simulink model "ScriptDemo"  (R2022b)
settings: configuration reference "TmVcThermal_Configuration_sub" (kept outside this file)
undefined symbols (not defined in the file or in its folder): aaaa, bbbb, cTmComprCtrl_D_u8HvacFlowTable_db, cTmComprCtrl_D_u8HvacFlowTable_sw, cTmComprCtrl_n_i16ChillCmpIMax, cTmComprCtrl_n_i16ChillCmpIMin, cTmComprCtrl_n_i16ChillCmpIMin666, cTmComprCtrl_n_i16ChillCmpPMax, cTmComprCtrl_n_i16ChillCmpPMin, cTmComprCtrl_n_i16CmpChillCoolRpmKiMax, cTmComprCtrl_n_i16CmpChillCoolRpmKiMin, cTmComprCtrl_n_i16CmpChillCoolRpmKpMax, cTmComprCtrl_n_i16CmpChillCoolRpmKpMin, cTmComprCtrl_n_i16CmpCoolRpmKiMax, cTmComprCtrl_n_i16CmpCoolRpmKiMin, cTmComprCtrl_n_i16CmpCoolRpmKpMax, cTmComprCtrl_n_i16CmpCoolRpmKpMin, cTmComprCtrl_n_i16SM4CmpHeatKiMax, cTmComprCtrl_n_i16SM4CmpHeatKiMin, cTmComprCtrl_n_i16SM4CmpHeatKpMax, cTmComprCtrl_n_i16SM4CmpHeatKpMin, cTmComprCtrl_n_i16SM5CmpHeatKiMax, cTmComprCtrl_n_i16SM5CmpHeatKiMin, cTmComprCtrl_n_i16SM5CmpHeatKpMax, cTmComprCtrl_n_i16SM5CmpHeatKpMin, cTmComprCtrl_n_i16SM6CmpHeatKiMax, cTmComprCtrl_n_i16SM6CmpHeatKiMin, cTmComprCtrl_n_i16SM6CmpHeatKpMax, cTmComprCtrl_n_i16SM6CmpHeatKpMin, cTmComprCtrl_n_u16CmpMaxSpdFanFltLimt, cTmComprCtrl_n_u16CmpMaxSpdLoSidePFltLimt, cTmComprCtrl_n_u16CmpMaxSpdSensorFltLimt, cTmComprCtrl_n_u16CompMinRpm, cTmComprCtrl_n_u16CompRpmIncThres, cTmComprCtrl_t_u16BattCooltFFPeriod, cTmComprCtrl_t_u16BattCooltPIPeriod, cTmComprCtrl_t_u16CmpCoolFFPeriod, cTmComprCtrl_t_u16CmpCoolPIPeriod, cTmComprCtrl_t_u16CoolCmpChillFFPeriod, cTmComprCtrl_t_u16CoolCmpChillPIPeriod, cTmComprCtrl_t_u16SM4CmpHeatFFPeriod, cTmComprCtrl_t_u16SM4CmpHeatPIPeriod, cTmComprCtrl_t_u16SM5CmpHeatFFPeriod, cTmComprCtrl_t_u16SM5CmpHeatPIPeriod, cTmComprCtrl_t_u16SM6CmpHeatFFPeriod, cTmComprCtrl_t_u16SM6CmpHeatPIPeriod, cTmComprCtrl_Te_EvapClearInteg, cTmComprCtrl_Te_i16HpReqTempSaturoffset, cTmComprCtrl_Te_i16SatLpReplaceDiff, cTmComprCtrl_Te_i16SM3BatDiffStartEvapDecOffset, cTmComprCtrl_Te_i16SM3EvapLo, cTmComprCtrl_Te_i16SM3TBatDiffEntEvapDecOffset, cTmComprCtrl_Te_i16SM3TBatDiffEntEvapDecOffsetQuit, cTmComprCtrl_Te_s32ErrCmpChillPIContinueCoolH, cTmComprCtrl_Te_s32ErrCmpChillPIContinueCoolL, cTmComprCtrl_Te_s32ErrCmpPIContinueChillH, cTmComprCtrl_Te_s32ErrCmpPIContinueChillL, cTmComprCtrl_Te_s32ErrCmpPIContinueCoolH, cTmComprCtrl_Te_s32ErrCmpPIContinueCoolL, cTmComprCtrl_Te_s32ErrCmpPIContinueHeatH ... (+398)
libraries: simulink x846, PCMULib x711, simulink_need_slupdate x4
(part 7 of 49)

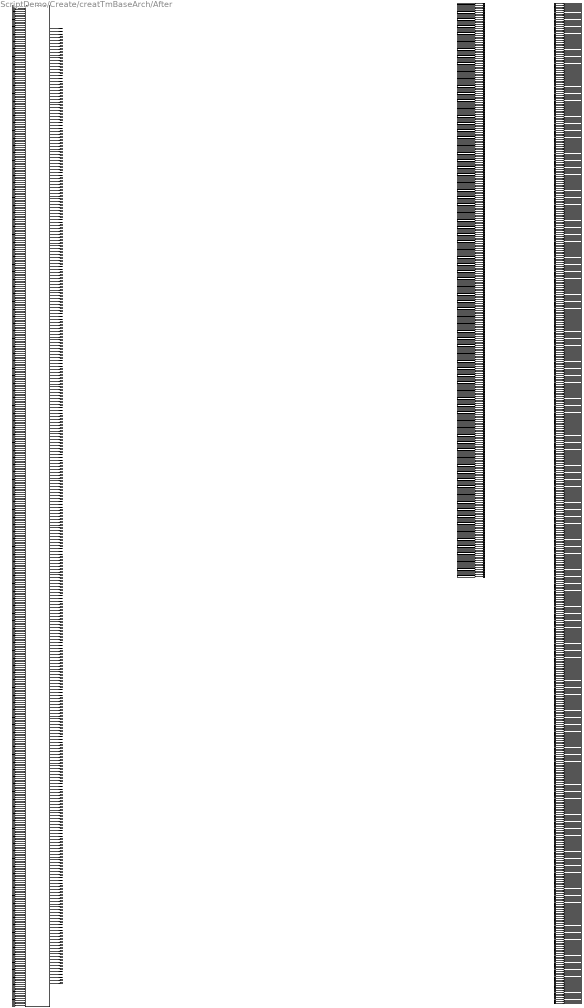
== system ScriptDemo/Create/creatTmBaseArch/After ==
  Ground{,1..567} (568 alike) : Ground
  Terminator{,1..325} (326 alike) : Terminator
  TmSwArch : ModelReference  ModelNameDialog=TmSwArch  ModelReferenceVersion=1.508
  wires:
  [sTmIn_L_s32WhlMotCooltFlowMinReq] -> TmSwArch/1
  [sTmIn_Te_s32WhlMotSysCooltT] -> TmSwArch/2
  [sTmIn_D_u8EradCoolReq] -> TmSwArch/3
  [sTmIn_Te_s32EradInvActl] -> TmSwArch/4
  [sTmIn_Te_s32EradWndgActl] -> TmSwArch/5
  [sTmIn_Tq_s32WhlMotSysTqEst] -> TmSwArch/6
  [sTmIn_D_u8DcdcCoolReq] -> TmSwArch/7
  [sTmIn_Te_s32DcdcActl] -> TmSwArch/8
  [sTmIn_L_s32DcDcMinCooltFlow] -> TmSwArch/9
  [sTmIn_D_u8ObcCoolReq] -> TmSwArch/10
  [sTmIn_D_u8OnBdChrgrHndlSts] -> TmSwArch/11
  [sTmIn_Te_s32ObcActl] -> TmSwArch/12
  [sTmIn_L_s32OnBdChrgrMinCooltFlow] -> TmSwArch/13
  [sTmIn_Te_s32OnBdChrgrCooltT] -> TmSwArch/14
  [sTmIn_Te_s32TDcDcCoolt] -> TmSwArch/15
  [sTmIn_D_u8HvBattCooltLvl] -> TmSwArch/16
  [sTmIn_D_u8DCChrgnHndlSts] -> TmSwArch/17
  [sTmIn_D_u8HvBattCoolgReq] -> TmSwArch/18
  [sTmIn_D_u8HvBattHeatgReq] -> TmSwArch/19
  [sTmIn_D_u8HvBattThermReq] -> TmSwArch/20
  [sTmIn_D_u16HVvBattLimnIndcn] -> TmSwArch/21
  [sTmIn_Pw_s32HvBattClimaPwr] -> TmSwArch/22
  [sTmIn_Te_s32BattHv] -> TmSwArch/23
  [sTmIn_Te_s32HvBattCooltT] -> TmSwArch/24
  [sTmIn_Te_s32HvBattCooltTReq] -> TmSwArch/25
  [sTmIn_L_s32HvBattCoolFlow1] -> TmSwArch/26
  [sTmIn_Te_s32HvBattCooltTOut] -> TmSwArch/27
  [sTmIn_L_s32IsgCooltFlowMinReq] -> TmSwArch/28
  [sTmIn_Te_s32Coolt] -> TmSwArch/29
  [sTmIn_D_u8HvgCoolReq] -> TmSwArch/30
  [sTmIn_Te_s32HvgInvActl] -> TmSwArch/31
  [sTmIn_Te_s32HvgWndgActl] -> TmSwArch/32
  [sTmIn_D_u8EngCooltLvl] -> TmSwArch/33
  [sTmIn_U_s32Sys] -> TmSwArch/34
  [sTmIn_D_u8UsgModSts1WdSts] -> TmSwArch/35
  [sTmIn_D_u8LVPwrSplyErrSts] -> TmSwArch/36
  [sTmIn_Z_s32RoadIncln] -> TmSwArch/37
  [sTmIn_D_u8CarModSts1] -> TmSwArch/38
  [sTmIn_Te_s32AmbTEstimd] -> TmSwArch/39
  [sTmIn_Te_s32Evap] -> TmSwArch/40
  [sTmIn_Te_s32EvapReq] -> TmSwArch/41
  [sTmIn_Te_s32HeadEstimdFirstRow] -> TmSwArch/42
  [sTmIn_Te_s32HeatrAirTReq] -> TmSwArch/43
  [sTmIn_Te_s32HvacHexAirT] -> TmSwArch/44
  [sTmIn_X_s32ClimtRcirc] -> TmSwArch/45
  [sTmIn_md_s32HexHeatrAirMFlowEstimd] -> TmSwArch/46
  [sTmIn_md_s32HvacAirMFlowEstimd] -> TmSwArch/47
  [yTmIn_B_AirCondEnbl] -> TmSwArch/48
  [yTmIn_B_ClimaDefrstSts] -> TmSwArch/49
  [yTmIn_B_HvacHeatgReq] -> TmSwArch/50
  [sTmIn_Te_s32IncarTemp] -> TmSwArch/51
  [yTmIn_B_AmbTEstimdQf] -> TmSwArch/52
  [sTmIn_D_u8IncarTempQf] -> TmSwArch/53
  [yTmIn_B_HvacOsaAndRecActrQfForHp] -> TmSwArch/54
  [yTmIn_B_TeEvap] -> TmSwArch/55
  [yTmIn_B_HvacHexAirTQf] -> TmSwArch/56
  [sTmIn_D_u8HvacFanSts] -> TmSwArch/57
  [yTmIn_B_ImpactDetect] -> TmSwArch/58
  [yTmIn_B_BattPmpOPflg] -> TmSwArch/59
  [yTmIn_B_BattPmpOPTF] -> TmSwArch/60
  [yTmIn_B_BattPmpSBflg] -> TmSwArch/61
  [yTmIn_B_BattPmpSBTF] -> TmSwArch/62
  [yTmIn_B_BattPmpSGflg] -> TmSwArch/63
  [yTmIn_B_BattPmpSGTF] -> TmSwArch/64
  [yTmIn_B_EmotPmpOPflg] -> TmSwArch/65
  [yTmIn_B_EmotPmpOPTF] -> TmSwArch/66
  [yTmIn_B_EmotPmpSBflg] -> TmSwArch/67
  [yTmIn_B_EmotPmpSBTF] -> TmSwArch/68
  [yTmIn_B_EmotPmpSGflg] -> TmSwArch/69
  [yTmIn_B_EmotPmpSGTF] -> TmSwArch/70
  [yTmIn_B_FanOutOPflg] -> TmSwArch/71
  [yTmIn_B_FanOutOPTF] -> TmSwArch/72
  [yTmIn_B_FanOutSBflg] -> TmSwArch/73
  [yTmIn_B_FanOutSBTF] -> TmSwArch/74
  [yTmIn_B_FanOutSGflg] -> TmSwArch/75
  [yTmIn_B_FanOutSGTF] -> TmSwArch/76
  [yTmIn_B_HmPumpOCflg] -> TmSwArch/77
  [yTmIn_B_HmPumpOCTF] -> TmSwArch/78
  [yTmIn_B_HmPumpSBflg] -> TmSwArch/79
  [yTmIn_B_HmPumpSBTF] -> TmSwArch/80
  [yTmIn_B_HmPumpSGflg] -> TmSwArch/81
  [yTmIn_B_HmPumpSGTF] -> TmSwArch/82
  [yTmIn_B_Sov1OPTF] -> TmSwArch/83
  [yTmIn_B_Sov1OPflg] -> TmSwArch/84
  [yTmIn_B_Sov1SBTF] -> TmSwArch/85
  [yTmIn_B_Sov1SBflg] -> TmSwArch/86
  [yTmIn_B_Sov1SGTF] -> TmSwArch/87
  [yTmIn_B_Sov1SGflg] -> TmSwArch/88
  [yTmIn_B_Sov2OPTF] -> TmSwArch/89
  [yTmIn_B_Sov2OPflg] -> TmSwArch/90
  [yTmIn_B_Sov2SBTF] -> TmSwArch/91
  [yTmIn_B_Sov2SBflg] -> TmSwArch/92
  [yTmIn_B_Sov2SGTF] -> TmSwArch/93
  [yTmIn_B_Sov2SGflg] -> TmSwArch/94
  [yTmIn_B_Sov3OPTF] -> TmSwArch/95
  [yTmIn_B_Sov3OPflg] -> TmSwArch/96
  [yTmIn_B_Sov3SBTF] -> TmSwArch/97
  [yTmIn_B_Sov3SBflg] -> TmSwArch/98
  [yTmIn_B_Sov3SGTF] -> TmSwArch/99
  [yTmIn_B_Sov3SGflg] -> TmSwArch/100
  [yTmIn_B_Sov4OPTF] -> TmSwArch/101
  [yTmIn_B_Sov4OPflg] -> TmSwArch/102
  [yTmIn_B_Sov4SBTF] -> TmSwArch/103
  [yTmIn_B_Sov4SBflg] -> TmSwArch/104
  [yTmIn_B_Sov4SGTF] -> TmSwArch/105
  [yTmIn_B_Sov4SGflg] -> TmSwArch/106
  [yTmIn_B_Sov5OPTF] -> TmSwArch/107
  [yTmIn_B_Sov5OPflg] -> TmSwArch/108
  [yTmIn_B_Sov5SBTF] -> TmSwArch/109
  [yTmIn_B_Sov5SBflg] -> TmSwArch/110
  [yTmIn_B_Sov5SGTF] -> TmSwArch/111
  [yTmIn_B_Sov5SGflg] -> TmSwArch/112
  [sTmIn_X_s32BattCooltPmpReq2F] -> TmSwArch/113
  [sTmIn_X_s32PTCPumpSpdReq2F] -> TmSwArch/114
  [sTmIn_D_u8CmprStsEnaReq2F] -> TmSwArch/115
  [sTmIn_n_s32CmprSpdReq2F] -> TmSwArch/116
  [sTmIn_Pw_s32CmprPwrEnaReq2F] -> TmSwArch/117
  [sTmIn_D_u8GrlShttrTrqBstReq2F] -> TmSwArch/118
  [sTmIn_D_u8BcfvVlvRefReq2F] -> TmSwArch/119
  [sTmIn_X_u8BcfvVlvPosReq2F] -> TmSwArch/120
  [sTmIn_D_u8BctvVlvRefReq2F] -> TmSwArch/121
  [sTmIn_X_u8BctvVlvPosReq2F] -> TmSwArch/122
  [yTmIn_B_BExvCalReq2F] -> TmSwArch/123
  [yTmIn_B_BExvMoveEnReq2F] -> TmSwArch/124
  [sTmIn_X_s32BExvPosnReq2F] -> TmSwArch/125
  [yTmIn_B_CExvCalReq2F] -> TmSwArch/126
  [yTmIn_B_CExvMoveEnaReq2F] -> TmSwArch/127
  [sTmIn_X_s32CExvPosnReq2F] -> TmSwArch/128
  [yTmIn_B_EctvVlvMoveEnaReq2F] -> TmSwArch/129
  [sTmIn_X_u8EctvVlvPosReq2F] -> TmSwArch/130
  [yTmIn_B_EExvCalReq2F] -> TmSwArch/131
  [yTmIn_B_EExvMoveEnaReq2F] -> TmSwArch/132
  [sTmIn_X_s32EExvPosnReq2F] -> TmSwArch/133
  [yTmIn_B_PtcEnaReq2F] -> TmSwArch/134
  [sTmIn_Pw_s32PtcPwrReq2F] -> TmSwArch/135
  [sTmIn_Te_s32PtcTReq2F] -> TmSwArch/136
  [sTmIn_L_s32PtcFlowReq2F] -> TmSwArch/137
  [sTmIn_X_s32FanPwmReq2F] -> TmSwArch/138
  [sTmIn_Z_s32VaneCtrlAngleReq2F] -> TmSwArch/139
  [sTmIn_X_s32EmCooltPmpReq2F] -> TmSwArch/140
  [yTmIn_B_HpmSov1ActvCmd2F] -> TmSwArch/141
  [yTmIn_B_HpmSov2ActvCmd2F] -> TmSwArch/142
  [yTmIn_B_HpmSov3ActvCmd2F] -> TmSwArch/143
  [yTmIn_B_EvaprVlvReqFrnt2F] -> TmSwArch/144
  [yTmIn_B_ChillerValveReq2F] -> TmSwArch/145
  [yTmIn_B_VaneCalEnbl2F] -> TmSwArch/146
  [yTmIn_B_HpmSov1Actv2FReq] -> TmSwArch/147
  [yTmIn_B_HpmSov2Actv2FReq] -> TmSwArch/148
  [yTmIn_B_HpmSov3Actv2FReq] -> TmSwArch/149
  [yTmIn_B_BattPmp2FReq] -> TmSwArch/150
  [yTmIn_B_PTCPumpSpd2FReq] -> TmSwArch/151
  [yTmIn_B_EvaprVlvFrnt2FReq] -> TmSwArch/152
  [yTmIn_B_CmprPwrEna2FReq] -> TmSwArch/153
  [yTmIn_B_CmprSpd2FReq] -> TmSwArch/154
  [yTmIn_B_CmprStsEna2FReq] -> TmSwArch/155
  [yTmIn_B_GrlShttrTrqBst2FReq] -> TmSwArch/156
  [yTmIn_B_BcfvVlvPos2FReq] -> TmSwArch/157
  [yTmIn_B_BcfvVlvRef2FReq] -> TmSwArch/158
  [yTmIn_B_BctvVlvPos2FReq] -> TmSwArch/159
  [yTmIn_B_BctvVlvRef2FReq] -> TmSwArch/160
  [yTmIn_B_BExvCal2FReq] -> TmSwArch/161
  [yTmIn_B_BExvMoveEna2FReq] -> TmSwArch/162
  [yTmIn_B_BExvPosn2FReq] -> TmSwArch/163
  [yTmIn_B_CExvCal2FReq] -> TmSwArch/164
  [yTmIn_B_CExvMoveEna2FReq] -> TmSwArch/165
  [yTmIn_B_CExvPosn2FReq] -> TmSwArch/166
  [yTmIn_B_ChillerValve2FReq] -> TmSwArch/167
  [yTmIn_B_EctvVlvMoveEna2FReq] -> TmSwArch/168
  [yTmIn_B_EctvVlvPos2FReq] -> TmSwArch/169
  [yTmIn_B_EExvCal2FReq] -> TmSwArch/170
  [yTmIn_B_EExvMoveEna2FReq] -> TmSwArch/171
  [yTmIn_B_EExvPosn2FReq] -> TmSwArch/172
  [yTmIn_B_PtcEna2FReq] -> TmSwArch/173
  [yTmIn_B_PtcFlow2FReq] -> TmSwArch/174
  [yTmIn_B_PtcPwr2FReq] -> TmSwArch/175
  [yTmIn_B_PtcT2FReq] -> TmSwArch/176
  [yTmIn_B_FanPwm2FReq] -> TmSwArch/177
  [yTmIn_B_VaneCalEnbl2FReq] -> TmSwArch/178
  [yTmIn_B_VaneCtrlAngle2FReq] -> TmSwArch/179
  [yTmIn_B_EmCooltPmp2FReq] -> TmSwArch/180
  [sTmIn_D_u8AcCmpr] -> TmSwArch/181
  [sTmIn_D_u8BattCoolLelIn] -> TmSwArch/182
  [sTmIn_D_u8EldtCoolLelIn] -> TmSwArch/183
  [sTmIn_D_u8ForHvacTyp] -> TmSwArch/184
  [sTmIn_D_u8HeatPump] -> TmSwArch/185
  [sTmIn_D_u8HvacRe] -> TmSwArch/186
  [sTmIn_D_u8Refrigerant] -> TmSwArch/187
  [sTmIn_D_u8ShutterConfig] -> TmSwArch/188
  [sTmIn_U_s32AcCompDischrgT] -> TmSwArch/189
  [sTmIn_U_s32AcCompInletT] -> TmSwArch/190
  [sTmIn_U_s32AcCondOutT] -> TmSwArch/191
  [sTmIn_U_s32AcEvapOutT] -> TmSwArch/192
  [sTmIn_U_s32AcIntelCondOutT] -> TmSwArch/193
  [sTmIn_U_s32HiSideP] -> TmSwArch/194
  [sTmIn_U_s32HiSidePNHP] -> TmSwArch/195
  [sTmIn_U_s32LoSideP] -> TmSwArch/196
  [sTmIn_U_s32CooltTSigForDtElec] -> TmSwArch/197
  [yTmIn_B_CPSRFbSt] -> TmSwArch/198
  [sTmIn_U_s32BattVolt] -> TmSwArch/199
  [yTmIn_B_HvBattThermModUD] -> TmSwArch/200
  [sTmIn_D_u8EexvBlkErr] -> TmSwArch/201
  [sTmIn_D_u8EexvElecStsErr] -> TmSwArch/202
  [sTmIn_D_u8EexvNVMFlt] -> TmSwArch/203
  [sTmIn_D_u8EexvOvrTempErr] -> TmSwArch/204
  [sTmIn_D_u8EexvVoltgRangErr] -> TmSwArch/205
  [sTmIn_D_u8EexvOvrTrvlErr] -> TmSwArch/206
  [sTmIn_D_u8CexvBlkErr] -> TmSwArch/207
  [sTmIn_D_u8CexvElecStsErr] -> TmSwArch/208
  [sTmIn_D_u8CexvNVMFlt] -> TmSwArch/209
  [sTmIn_D_u8CexvOvrTempErr] -> TmSwArch/210
  [sTmIn_D_u8CexvVoltgRangErr] -> TmSwArch/211
  [sTmIn_D_u8CexvOvrTrvlErr] -> TmSwArch/212
  [sTmIn_D_u8EctvFaultSts] -> TmSwArch/213
  [sTmIn_D_u8EctvTempSts] -> TmSwArch/214
  [sTmIn_D_u8EctvVoltSts] -> TmSwArch/215
  [sTmIn_D_u8BexvBlkErr] -> TmSwArch/216
  [sTmIn_D_u8BexvCalibSts] -> TmSwArch/217
  [sTmIn_D_u8BexvElecStsErr] -> TmSwArch/218
  [sTmIn_D_u8BexvNVMFlt] -> TmSwArch/219
  [sTmIn_D_u8BexvOvrTempErr] -> TmSwArch/220
  [sTmIn_D_u8BexvOvrTrvlErr] -> TmSwArch/221
  [sTmIn_D_u8BexvPreHeatgSts] -> TmSwArch/222
  [sTmIn_D_u8BexvVoltgRangErr] -> TmSwArch/223
  [sTmIn_X_s32BexvPosSts] -> TmSwArch/224
  [yTmIn_B_BexvComFault] -> TmSwArch/225
  [sTmIn_D_u8BcfvFaultSts] -> TmSwArch/226
  [sTmIn_D_u8BcfvNVMFlt] -> TmSwArch/227
  [sTmIn_D_u8BcfvTempSts] -> TmSwArch/228
  [sTmIn_D_u8BcfvVoltSts] -> TmSwArch/229
  [sTmIn_D_u8BctvFaultSts] -> TmSwArch/230
  [sTmIn_D_u8BctvNVMFlt] -> TmSwArch/231
  [sTmIn_D_u8BctvTempSts] -> TmSwArch/232
  [sTmIn_D_u8BctvVoltSts] -> TmSwArch/233
  [sTmIn_X_s32BctvPosSts] -> TmSwArch/234
  [sTmIn_D_u8CmprRAMFault] -> TmSwArch/235
  [sTmIn_D_u8CmprROMFault] -> TmSwArch/236
  [sTmIn_D_u8CmprRotorLockStat] -> TmSwArch/237
  [sTmIn_D_u8CmprSts1] -> TmSwArch/238
  [sTmIn_D_u8HVoltResonanceStat] -> TmSwArch/239
  [sTmIn_D_u8InCurrOverCurrStat] -> TmSwArch/240
  [sTmIn_D_u8LiquidSluggingStat] -> TmSwArch/241
  [sTmIn_D_u8MotorCurrOverCurrStat] -> TmSwArch/242
  [sTmIn_D_u8OverMotorCurrStat] -> TmSwArch/243
  [sTmIn_D_u8OverPowerStat] -> TmSwArch/244
  [sTmIn_I_s32ElacCmprHvActl] -> TmSwArch/245
  [sTmIn_n_s32ElacCmprActl] -> TmSwArch/246
  [sTmIn_Te_s32CmprT1] -> TmSwArch/247
  [sTmIn_U_s32ElacCmprHvActl] -> TmSwArch/248
  [sTmIn_D_u8ErrRespAGM] -> TmSwArch/249
  [sTmIn_D_u8GrlActTrqBoost] -> TmSwArch/250
  [sTmIn_D_u8GrlHldTrqActive] -> TmSwArch/251
  [sTmIn_D_u8GrlShttrMoveActive] -> TmSwArch/252
  [sTmIn_D_u8GrlShttrNVMFlt] -> TmSwArch/253
  [sTmIn_D_u8GrlShttrOvertravelErr] -> TmSwArch/254
  [sTmIn_D_u8GrlShttrOverVolt] -> TmSwArch/255
  [sTmIn_D_u8GrlShttrStsShttrActrFlt] -> TmSwArch/256
  [sTmIn_D_u8GrlShttrStsShttrBlkd] -> TmSwArch/257
  [sTmIn_D_u8GrlShttrStsShttrCalActv] -> TmSwArch/258
  [sTmIn_D_u8GrlShttrStsShttrCalIndcd] -> TmSwArch/259
  [sTmIn_D_u8GrlShttrStsShttrElecErr] -> TmSwArch/260
  [sTmIn_D_u8GrlShttrStsShttrSnsrFlt] -> TmSwArch/261
  [sTmIn_D_u8GrlShttrStsShttrTErr] -> TmSwArch/262
  [sTmIn_D_u8GrlShttrStsShttrULoErr] -> TmSwArch/263
  [sTmIn_X_s32GrlShttrStsShttrPosnRaw] -> TmSwArch/264
  [sTmIn_D_u8CircForDrvrShoOrOpen] -> TmSwArch/265
  [sTmIn_D_u8CooltTInSnsrFlt] -> TmSwArch/266
  [sTmIn_D_u8CooltTOutOfRng] -> TmSwArch/267
  [sTmIn_D_u8CooltTOutSnsrFlt] -> TmSwArch/268
  [sTmIn_D_u8HeatrStsSig] -> TmSwArch/269
  [sTmIn_D_u8HvOutOfRng] -> TmSwArch/270
  [sTmIn_D_u8ICnsOutOfRng] -> TmSwArch/271
  [sTmIn_D_u8MemErr] -> TmSwArch/272
  [sTmIn_D_u8SelfTmpSigHwProtn] -> TmSwArch/273
  [sTmIn_D_u8SelfTmpSigOvrheatg] -> TmSwArch/274
  [sTmIn_D_u8TInMtrlSnsrFlt] -> TmSwArch/275
  [sTmIn_D_u8ULoOutOfRng] -> TmSwArch/276
  [sTmIn_Pw_s32HvHeatrPwrCns] -> TmSwArch/277
  [sTmIn_Pw_s32HvHeatrPwrCnsDes] -> TmSwArch/278
  [sTmIn_Te_s32WtrTInIntk] -> TmSwArch/279
  [sTmIn_Te_s32WtrTInOutl] -> TmSwArch/280
  [sTmIn_D_u8SrvRqrd] -> TmSwArch/281
  [sTmIn_D_u8TmpSigProtnOfSelfTmp] -> TmSwArch/282
  [sTmIn_D_u8HvCoolgCmd] -> TmSwArch/283
  [sTmIn_D_u8HvHvacCmd] -> TmSwArch/284
  [sTmIn_D_u8HvActvSts] -> TmSwArch/285
  [sTmIn_D_u8PowerPackStatus] -> TmSwArch/286
  [sTmIn_Pw_s32HvCoolgAllwd] -> TmSwArch/287
  [sTmIn_Pw_s32HvHeatgAllwd] -> TmSwArch/288
  [yTmIn_B_ElAcEnable] -> TmSwArch/289
  [yTmIn_B_HvCooltHeatrEnad] -> TmSwArch/290
  [sTmIn_v_s32VehSpdLgt] -> TmSwArch/291
  [yTmIn_B_StarDiagEval] -> TmSwArch/292
  [sTmIn_D_u8HvActvReq] -> TmSwArch/293
  [sTmIn_D_u8DCChrgSt] -> TmSwArch/294
  [yTmIn_B_NOPCoolReq] -> TmSwArch/295
  [sTmIn_Pw_s32HvBattChrgnPwrCritDes1] -> TmSwArch/296
  [yTmIn_B_ChargePsr] -> TmSwArch/297
  [sTmIn_Te_s32BattHvMin] -> TmSwArch/298
  [sTmIn_D_u8HvBattSupChrgThermSts] -> TmSwArch/299
  [sTmIn_D_u8OnBdChrgrSt] -> TmSwArch/300
  [sTmIn_D_u8DistHvBatt] -> TmSwArch/301
  [sTmIn_D_u8ElecDriveline] -> TmSwArch/302
  [sTmIn_D_u8HiWayAsst] -> TmSwArch/303
  [sTmIn_D_u8CruiseCtrl] -> TmSwArch/304
  [sTmIn_D_u8BattCntct] -> TmSwArch/305
  [sTmIn_U_s32HvBattUDc] -> TmSwArch/306
  [yTmIn_B_EvaprTFrntUD] -> TmSwArch/307
  [sTmIn_Te_s32HmiCmptmtTSpForRowFirstRi] -> TmSwArch/308
  [sTmIn_Te_s32HmiCmptmtTSpForRowFirstLe] -> TmSwArch/309
  [sTmIn_D_u8HvUSplyErrSts] -> TmSwArch/310
  [sTmIn_D_u8LnchModSts] -> TmSwArch/311
  [sTmIn_D_u8LaunchCtrl] -> TmSwArch/312
  [sTmIn_X_s32HvacTFlpActlPosnFrtRowLe] -> TmSwArch/313
  [sTmIn_X_s32HvacTFlpActlPosnFrtRowRi] -> TmSwArch/314
  [sTmIn_D_u8HmiCmptmtTSpSpclForRowFirstLe] -> TmSwArch/315
  [sTmIn_D_u8HmiCmptmtTSpSpclForRowFirstRi] -> TmSwArch/316
  [sTmIn_D_u8SysQf] -> TmSwArch/317
  [yTmIn_B_ErrRespHVCH] -> TmSwArch/318
  [sTmIn_I_s32HeatrICnsSig] -> TmSwArch/319
  [sTmIn_D_u8HeatrInfoCompProtn] -> TmSwArch/320
  [sTmIn_U_u8SplyUForCtrlUnitVal] -> TmSwArch/321
  [sTmIn_D_u8SelfSigProOfTmpResd] -> TmSwArch/322
  [sTmIn_D_u8ResdForSnsrFlt] -> TmSwArch/323
  [sTmIn_D_u8SrvRqrdResd] -> TmSwArch/324
  [sTmIn_D_u8FltInComHVCH] -> TmSwArch/325
  [sTmIn_D_u8FltPrsnt] -> TmSwArch/326
  [sTmIn_D_u8FltPrsntResd] -> TmSwArch/327
  [yTmIn_B_EctvComFault] -> TmSwArch/328
  [sTmIn_D_u8EctvPosSts] -> TmSwArch/329
  [sTmIn_D_u8EctvRunSts] -> TmSwArch/330
  [sTmIn_D_u8EctvSpdLvl] -> TmSwArch/331
  [yTmIn_B_BctvComFault] -> TmSwArch/332
  [sTmIn_D_u8BctvVlvMode] -> TmSwArch/333
  [sTmIn_D_u8BctvRunSts] -> TmSwArch/334
  [sTmIn_D_u8BctvSpdLvl] -> TmSwArch/335
  [yTmIn_B_BcfvComFault] -> TmSwArch/336
  [sTmIn_D_u8BcfvVlvMode] -> TmSwArch/337
  [sTmIn_X_s32BcfvPosSts] -> TmSwArch/338
  [sTmIn_D_u8BcfvRunSts] -> TmSwArch/339
  [sTmIn_D_u8BcfvSpdLvl] -> TmSwArch/340
  [sTmIn_D_u8ErrRespACCM] -> TmSwArch/341
  [sTmIn_D_u8SpdErrSts] -> TmSwArch/342
  [sTmIn_D_u8CtrlrErrSts] -> TmSwArch/343
  [sTmIn_D_u8AccmDrvrSircSnErrStsts] -> TmSwArch/344
  [sTmIn_D_u8DrvrSircSnstPlausErrSts] -> TmSwArch/345
  [sTmIn_D_u8AccmHvSnsrU1ErrSts] -> TmSwArch/346
  [sTmIn_D_u8AccmHvSnsrU2ErrSts] -> TmSwArch/347
  [sTmIn_D_u8AccmHvSnsrIErrSts] -> TmSwArch/348
  [sTmIn_D_u8AccmSnsrICrctErrSts] -> TmSwArch/349
  [sTmIn_D_u8HvSnsrIPlausErrSts] -> TmSwArch/350
  [sTmIn_D_u8HvSnsrUPlausErrSts] -> TmSwArch/351
  [sTmIn_D_u8AccmPhaseWireErrSts] -> TmSwArch/352
  [sTmIn_D_u8AccmT1ErrSts] -> TmSwArch/353
  [sTmIn_D_u8AccmT2ErrSts] -> TmSwArch/354
  [sTmIn_D_u8AccmCmprTOperErr1] -> TmSwArch/355
  [sTmIn_D_u8AccmCmprTOperErr2] -> TmSwArch/356
  [sTmIn_D_u8TPlausErrSts] -> TmSwArch/357
  [sTmIn_D_u8AccmLoUSplyErrSts] -> TmSwArch/358
  [sTmIn_I_s32CmprFbCmprIPha] -> TmSwArch/359
  [sTmIn_D_u8CmprSts2] -> TmSwArch/360
  [sTmIn_Te_s32CmprT2] -> TmSwArch/361
  [sTmIn_D_u8EEPROMFault] -> TmSwArch/362
  [sTmIn_D_u8LostCommStat] -> TmSwArch/363
  [sTmIn_D_u8CmprSpdIncrReq] -> TmSwArch/364
  [sTmIn_D_u8BexvMovSts] -> TmSwArch/365
  [yTmIn_B_CexvComFault] -> TmSwArch/366
  [sTmIn_X_s32CexvPosSts] -> TmSwArch/367
  [sTmIn_D_u8CexvCalibSts] -> TmSwArch/368
  [sTmIn_D_u8CexvMovSts] -> TmSwArch/369
  [sTmIn_D_u8CexvPreHeatgSts] -> TmSwArch/370
  [yTmIn_B_EexvComFault] -> TmSwArch/371
  [sTmIn_X_s32EexvPosSts] -> TmSwArch/372
  [sTmIn_D_u8EexvCalibSts] -> TmSwArch/373
  [sTmIn_D_u8EexvMovSts] -> TmSwArch/374
  [sTmIn_D_u8EexvPreHeatgSts] -> TmSwArch/375
  [yTmIn_B_HvacHexAirTUD] -> TmSwArch/376
  [yTmIn_B_EcoClimaSts] -> TmSwArch/377
  [sTmIn_t_s32BattPmpPwmTHigh] -> TmSwArch/378
  [yTmIn_B_BattPmpTHighValid] -> TmSwArch/379
  [sTmIn_t_s32BattPmpPwmTLow] -> TmSwArch/380
  [yTmIn_B_BattPmpTLowValid] -> TmSwArch/381
  [sTmIn_t_s32EmotPmpPwmTHigh] -> TmSwArch/382
  [yTmIn_B_EmotPmpTHighValid] -> TmSwArch/383
  [sTmIn_t_s32EmotPmpPwmTLow] -> TmSwArch/384
  [yTmIn_B_EmotPmpTLowValid] -> TmSwArch/385
  [sTmIn_t_s32FanPwmTHigh] -> TmSwArch/386
  [yTmIn_B_FanTHighValid] -> TmSwArch/387
  [sTmIn_t_s32FanPwmTLow] -> TmSwArch/388
  [yTmIn_B_FanTLowValid] -> TmSwArch/389
  [sTmIn_t_s32HmPumpPwmTHigh] -> TmSwArch/390
  [yTmIn_B_HmPumpTHighValid] -> TmSwArch/391
  [sTmIn_t_s32HmPumpPwmTLow] -> TmSwArch/392
  [yTmIn_B_HmPumpTLowValid] -> TmSwArch/393
  [sTmIn_D_u8HeatStopReq] -> TmSwArch/394
  [yTmIn_B_AD4CoolReq] -> TmSwArch/395
  [sTmIn_L_s32AD4CooltFlowReq] -> TmSwArch/396
  [sTmIn_L_s32DHUCooltFlowMinReq] -> TmSwArch/397
  [sTmIn_D_u8VcEvLoSidePOP] -> TmSwArch/398
  [sTmIn_D_u8VcEvLoSidePSB] -> TmSwArch/399
  [sTmIn_D_u8VcEvHiSidePOP] -> TmSwArch/400
  [sTmIn_D_u8VcEvHiSidePSB] -> TmSwArch/401
  [sTmIn_D_u8VcEvHiSideTmpSnrSG] -> TmSwArch/402
  [sTmIn_D_u8VcEvOutrCondOutTOP] -> TmSwArch/403
  [sTmIn_D_u8VcEvChillerOutTSG] -> TmSwArch/404
  [sTmIn_D_u8VcEvChillerOutTOP] -> TmSwArch/405
  [sTmIn_D_u8VcEvInrCondOutTSG] -> TmSwArch/406
  [sTmIn_D_u8VcEvInrCondOutTOP] -> TmSwArch/407
  [sTmIn_D_u8VcEvEvapOutTSG] -> TmSwArch/408
  [sTmIn_D_u8VcEvEvapOutTOP] -> TmSwArch/409
  [sTmIn_D_u8VcEvCmprDischrgTSG] -> TmSwArch/410
  [sTmIn_D_u8VcEvCmprDischrgTOP] -> TmSwArch/411
  [sTmIn_D_u8VcEvTmpClSrSG] -> TmSwArch/412
  [sTmIn_D_u8VcEvTmpClSrOP] -> TmSwArch/413
  [sTmIn_D_u8VcEvBattCooltLvlLo] -> TmSwArch/414
  [sTmIn_D_u8VcEvNoHpHighSidePSnrOP] -> TmSwArch/415
  [sTmIn_D_u8VcEvNoHpHighSidePSnrSB] -> TmSwArch/416
  [sTmIn_D_u8VcEvSov1OP] -> TmSwArch/417
  [sTmIn_D_u8VcEvSov1SB] -> TmSwArch/418
  [sTmIn_D_u8VcEvSov1SG] -> TmSwArch/419
  [sTmIn_D_u8VcEvSov2OP] -> TmSwArch/420
  [sTmIn_D_u8VcEvSov2SB] -> TmSwArch/421
  [sTmIn_D_u8VcEvSov2SG] -> TmSwArch/422
  [sTmIn_D_u8VcEvSov3OP] -> TmSwArch/423
  [sTmIn_D_u8VcEvSov3SB] -> TmSwArch/424
  [sTmIn_D_u8VcEvSov3SG] -> TmSwArch/425
  [sTmIn_D_u8VcEvSov4OP] -> TmSwArch/426
  [sTmIn_D_u8VcEvSov4SB] -> TmSwArch/427
  [sTmIn_D_u8VcEvSov4SG] -> TmSwArch/428
  [sTmIn_D_u8VcEvSov5OP] -> TmSwArch/429
  [sTmIn_D_u8VcEvSov5SB] -> TmSwArch/430
  [sTmIn_D_u8VcEvSov5SG] -> TmSwArch/431
  [sTmIn_D_u8VcEvSBFan] -> TmSwArch/432
  [sTmIn_D_u8VcEvSGFan] -> TmSwArch/433
  [sTmIn_D_u8VcEvOPFan] -> TmSwArch/434
  [sTmIn_D_u8VcEvFanOvrTShDwn] -> TmSwArch/435
  [sTmIn_D_u8VcEvBlokFan] -> TmSwArch/436
  [sTmIn_D_u8VcEvCircutInteFlt] -> TmSwArch/437
  [sTmIn_D_u8VcEvVolErrFan] -> TmSwArch/438
  [sTmIn_D_u8VcEvHmPumpSG] -> TmSwArch/439
  [sTmIn_D_u8VcEvHmPumpSB] -> TmSwArch/440
  [sTmIn_D_u8VcEvHmPumpOC] -> TmSwArch/441
  [sTmIn_D_u8VcEvHmPmpOvrTShutDwn] -> TmSwArch/442
  [sTmIn_D_u8VcEvHmPmpStall] -> TmSwArch/443
  [sTmIn_D_u8VcEvHmPmpVolErr] -> TmSwArch/444
  [sTmIn_D_u8VcEvHmPmpDyRn] -> TmSwArch/445
  [sTmIn_D_u8VcEvSGBatteryPmp] -> TmSwArch/446
  [sTmIn_D_u8VcEvSBBatteryPmp] -> TmSwArch/447
  [sTmIn_D_u8VcEvOCBatteryPmp] -> TmSwArch/448
  [sTmIn_D_u8VcEvBattPmpOvrTShutDwn] -> TmSwArch/449
  [sTmIn_D_u8VcEvBattPmpStall] -> TmSwArch/450
  [sTmIn_D_u8VcEvBattPmpVolErr] -> TmSwArch/451
  [sTmIn_D_u8VcEvBattPmpDyn] -> TmSwArch/452
  [sTmIn_D_u8VcEvSGEmotor] -> TmSwArch/453
  [sTmIn_D_u8VcEvSBEmotor] -> TmSwArch/454
  [sTmIn_D_u8VcEvOCEmotor] -> TmSwArch/455
  [sTmIn_D_u8VcEvEmPmpOvrTShutDwn] -> TmSwArch/456
  [sTmIn_D_u8VcEvEmPmpStall] -> TmSwArch/457
  [sTmIn_D_u8VcEvEmPmpVolErr] -> TmSwArch/458
  [sTmIn_D_u8VcEvEmPmpDyRn] -> TmSwArch/459
  [sTmIn_D_u8VcEvBctvOthrErr] -> TmSwArch/460
  [sTmIn_D_u8VcEvFltTemBCTV] -> TmSwArch/461
  [sTmIn_D_u8VcEvBctvBlk] -> TmSwArch/462
  [sTmIn_D_u8VcEvBctvErrResp] -> TmSwArch/463
  [sTmIn_D_u8VcEvFltVolBCTV] -> TmSwArch/464
  [sTmIn_D_u8VcEvBctvNVMFlt] -> TmSwArch/465
  [sTmIn_D_u8VcEvBctvIniFail] -> TmSwArch/466
  [sTmIn_D_u8VcEvBcfvOthrErr] -> TmSwArch/467
  [sTmIn_D_u8VcEvFltTempBCFV] -> TmSwArch/468
  [sTmIn_D_u8VcEvBcfvBlk] -> TmSwArch/469
  [sTmIn_D_u8VcEvBcfvErrResp] -> TmSwArch/470
  [sTmIn_D_u8VcEvFltVolBCFV] -> TmSwArch/471
  [sTmIn_D_u8VcEvBcfvNVMFlt] -> TmSwArch/472
  [sTmIn_D_u8VcEvBcfvIniFail] -> TmSwArch/473
  [sTmIn_D_u8VcEvEctvDrvMotorFlt] -> TmSwArch/474
  [sTmIn_D_u8VcEvWarnECRV] -> TmSwArch/475
  [sTmIn_D_u8VcEvEcrvErrResp] -> TmSwArch/476
  [sTmIn_D_u8VcEvFltVolECRV] -> TmSwArch/477
  [sTmIn_D_u8VcEvBexvIniFail] -> TmSwArch/478
  [sTmIn_D_u8VcEvBexvOvrTempErr] -> TmSwArch/479
  [sTmIn_D_u8VcEvBexvBlkErr] -> TmSwArch/480
  [sTmIn_D_u8VcEvBexvErrResp] -> TmSwArch/481
  [sTmIn_D_u8VcEvBexvVoltgRangErr] -> TmSwArch/482
  [sTmIn_D_u8VcEvBexvNVMFlt] -> TmSwArch/483
  [sTmIn_D_u8VcEvCexvIniFail] -> TmSwArch/484
  [sTmIn_D_u8VcEvCexvOvrTempErr] -> TmSwArch/485
  [sTmIn_D_u8VcEvCexvBlkErr] -> TmSwArch/486
  [sTmIn_D_u8VcEvCexvErrResp] -> TmSwArch/487
  [sTmIn_D_u8VcEvCexvVoltgRangErr] -> TmSwArch/488
  [sTmIn_D_u8VcEvCexvNVMFlt] -> TmSwArch/489
  [sTmIn_D_u8VcEvEexvIniFail] -> TmSwArch/490
  [sTmIn_D_u8VcEvEexvOvrTempErr] -> TmSwArch/491
  [sTmIn_D_u8VcEvEexvBlkErr] -> TmSwArch/492
  [sTmIn_D_u8VcEvEexvErrResp] -> TmSwArch/493
  [sTmIn_D_u8VcEvEexvVoltgRangErr] -> TmSwArch/494
  [sTmIn_D_u8VcEvEexvNVMFlt] -> TmSwArch/495
  [sTmIn_D_u8VcEvAccmUSplyErr] -> TmSwArch/496
  [sTmIn_D_u8VcEvAccmOCFlt] -> TmSwArch/497
  [sTmIn_D_u8VcEvAccmMotOvrCur] -> TmSwArch/498
  [sTmIn_D_u8VcEvAccmComFlt] -> TmSwArch/499
  [sTmIn_D_u8VcEvCurDrCirtACCM] -> TmSwArch/500
  [sTmIn_D_u8VcEvAccmRotorLock] -> TmSwArch/501
  [sTmIn_D_u8VcEvAccmOPFlt] -> TmSwArch/502
  [sTmIn_D_u8VcEvLiquidSluggingACCM] -> TmSwArch/503
  [sTmIn_D_u8VcEvMemFltAccm] -> TmSwArch/504
  [sTmIn_D_u8VcEvTM_AGM_OVRTEMP] -> TmSwArch/505
  [sTmIn_D_u8VcEvAgsBlk] -> TmSwArch/506
  [sTmIn_D_u8VcEvAgsErrResp] -> TmSwArch/507
  [sTmIn_D_u8VcEvAgsVoltErr] -> TmSwArch/508
  [sTmIn_D_u8VcEvAgsMechErr] -> TmSwArch/509
  [sTmIn_D_u8VcEvAgsNVMFlt] -> TmSwArch/510
  [sTmIn_D_u8VcEvAgsElecErr] -> TmSwArch/511
  [sTmIn_D_u8VcEvIGBTSpOrOpHVCH] -> TmSwArch/512
  [sTmIn_D_u8VcEvLoVoOvrHVCH] -> TmSwArch/513
  [sTmIn_D_u8VcEvVolMemErrHVCH] -> TmSwArch/514
  [sTmIn_D_u8VcEvComFltHVCH] -> TmSwArch/515
  [sTmIn_D_u8VcEvHiVoOvrHVCH] -> TmSwArch/516
  [sTmIn_D_u8VcEvCoolTempOutOfRng] -> TmSwArch/517
  [sTmIn_D_u8VcEvTempSerIntHVCH] -> TmSwArch/518
  [sTmIn_D_u8VcEvTempSerOutHVCH] -> TmSwArch/519
  [sTmIn_D_u8VcEvHWProtHVCH] -> TmSwArch/520
  [sTmIn_D_u8VcEvInterSerTempHVCH] -> TmSwArch/521
  [sTmIn_D_u8VcEvCurrOutOfRng] -> TmSwArch/522
  [sTmIn_D_u8LackRefrigerant] -> TmSwArch/523
  [sTmIn_D_u8HvBoostMod] -> TmSwArch/524
  [yTmIn_B_HmiMaxACReq] -> TmSwArch/525
  [yTmIn_B_GrlShttrAutoCalibReq2FReq] -> TmSwArch/526
  [yTmIn_B_GrlShttrAutoCalibReqReq2F] -> TmSwArch/527
  [sTmIn_X_s32PTCPumpPwmFb] -> TmSwArch/528
  [yTmIn_B_MessMissBctv] -> TmSwArch/529
  [yTmIn_B_MessMissBCFV] -> TmSwArch/530
  [yTmIn_B_MessMissECRV] -> TmSwArch/531
  [yTmIn_B_MessMissBEXV] -> TmSwArch/532
  [yTmIn_B_MessMissCEXV] -> TmSwArch/533
  [yTmIn_B_MessMissEEXV] -> TmSwArch/534
  [yTmIn_B_MessMissAccm] -> TmSwArch/535
  [yTmIn_B_MessMissAGM] -> TmSwArch/536
  [yTmIn_B_MessMissHVCH] -> TmSwArch/537
  [sTmIn_Tq_s32TotAxle] -> TmSwArch/538
  [sTmIn_Z_s32HvacModResp] -> TmSwArch/539
  [sTmIn_Te_s32HvBattTAvg] -> TmSwArch/540
  [yTmIn_B_AD4CoolReqForBkp] -> TmSwArch/541
  [sTmIn_L_s32AD4CooltFlowReqForBkp] -> TmSwArch/542
  [yTmIn_B_ChillerValveReqFb] -> TmSwArch/543
  [yTmIn_B_EvaprVlvReqFrntFb] -> TmSwArch/544
  [yTmIn_B_HpmSov1ActvCmdFb] -> TmSwArch/545
  [yTmIn_B_HpmSov2ActvCmdFb] -> TmSwArch/546
  [yTmIn_B_HpmSov3ActvCmdFb] -> TmSwArch/547
  [yTmIn_B_EmActivHeatAllwd] -> TmSwArch/548
  [sTmIn_D_u8IsgHeatFdBck] -> TmSwArch/549
  [sTmIn_D_u8WhlMotSysHeatFdBck] -> TmSwArch/550
  [sTmIn_Pw_s32IsgHeatPwrAct] -> TmSwArch/551
  [sTmIn_Pw_s32WhlMotSysHeatPwrAct] -> TmSwArch/552
  [sTmIn_Pw_s32ElecDrvHeatgPwrAllwd] -> TmSwArch/553
  [sTmIn_Pw_s32WhlMotSysHeatPwrMax] -> TmSwArch/554
  [sTmIn_Pw_s32IsgHeatPwrMax] -> TmSwArch/555
  [sTmIn_X_s32BattCooltPmpPwmFb] -> TmSwArch/556
  [sTmIn_D_u8CmprSupplrNo] -> TmSwArch/557
  [sTmIn_D_u8VcEvEctvBlk] -> TmSwArch/558
  [sTmIn_D_u8VcEvOVACCM] -> TmSwArch/559
  [sTmIn_D_u8VcEvAccmIgbtOvrTErr] -> TmSwArch/560
  [sTmIn_D_u8VcEvAccmSnsrFlt] -> TmSwArch/561
  [sTmIn_D_u8VcEvAccmPhaseFail] -> TmSwArch/562
  [yTmIn_B_AD4CoolReqForBkpUD] -> TmSwArch/563
  [yTmIn_B_AD4CoolReqUD] -> TmSwArch/564
  [yTmIn_B_AD4CooltFlowReqForBkpUD] -> TmSwArch/565
  [yTmIn_B_AD4CooltFlowReqUD] -> TmSwArch/566
  [sTmIn_D_u8VcEvOvrTempHVCH] -> TmSwArch/567
  [sTmIn_B_HvBattLimnIndcnUD] -> TmSwArch/568
  TmSwArch/1 -> [sTmOut_n_u16ElacCmprReq]
  TmSwArch/2 -> [sTmOut_D_u8ElacCmprRelease]
  TmSwArch/3 -> [sTmOut_Pw_s32ElacCmprMax]
  TmSwArch/4 -> [sTmOut_X_s32EexvVlvPosReq]
  TmSwArch/5 -> [yTmOut_B_EexvPosnCalibReq]
  TmSwArch/6 -> [yTmOut_B_EexvPosnMovEnable]
  TmSwArch/7 -> [sTmOut_X_s32BexvVlvPosReq]
  TmSwArch/8 -> [yTmOut_B_BexvPosnCalibReq]
  TmSwArch/9 -> [yTmOut_B_BexvPosnMovEnable]
  TmSwArch/10 -> [sTmOut_X_s32CexvVlvPosReq]
  TmSwArch/11 -> [yTmOut_B_CexvPosnCalibReq]
  TmSwArch/12 -> [yTmOut_B_CexvPosnMovEnable]
  TmSwArch/13 -> [sTmOut_D_u8BctvVlvRefDrvReq]
  TmSwArch/14 -> [sTmOut_X_u8BctvVlvPosReq]
  TmSwArch/15 -> [sTmOut_D_u8BcfvVlvRefDrvReq]
  TmSwArch/16 -> [sTmOut_X_u8BcfvVlvPosReq]
  TmSwArch/17 -> [yTmOut_B_EctvVlvMovEna]
  TmSwArch/18 -> [sTmOut_D_u8EctvVlvPosReq]
  TmSwArch/19 -> [sTmOut_Te_s32PTCTempReq]
  TmSwArch/20 -> [sTmOut_Z_s32PTCCoolantFlowrate]
  TmSwArch/21 -> [sTmOut_Pw_s32PTCPowerAlld]
  TmSwArch/22 -> [yTmOut_B_PTCEnabled]
  TmSwArch/23 -> [yTmOut_B_VaneCalEnbl]
  TmSwArch/24 -> [sTmOut_Z_s32VaneCtrlAngleReq]
  TmSwArch/25 -> [sTmOut_D_u8GrlShttrTrqBstReq]
  TmSwArch/26 -> [sTmOut_D_u8Sov1OnOffSts]
  TmSwArch/27 -> [sTmOut_D_u8Sov2OnOffSts]
  TmSwArch/28 -> [sTmOut_D_u8AirCondCmpsrStats]
  TmSwArch/29 -> [sTmOut_t_u32CmprRunTime]
  TmSwArch/30 -> [yTmOut_B_CoolgLimd]
  TmSwArch/31 -> [sTmOut_D_u8CoolgLoad]
  TmSwArch/32 -> [sTmOut_X_s32PTCPumpSpdReq]
  TmSwArch/33 -> [sTmOut_Pw_s32HtrPmpPwrCns]
  TmSwArch/34 -> [sTmOut_Pw_s32HvBattPmpPwrCns]
  TmSwArch/35 -> [sTmOut_Pw_s32EldtPmpPwrCns]
  TmSwArch/36 -> [sTmOut_n_s32HeatrPmpSpdAct]
  TmSwArch/37 -> [sTmOut_Pw_s32FanPwrCns]
  TmSwArch/38 -> [sTmOut_D_u8ResrvdSigForCCM1]
  TmSwArch/39 -> [sTmOut_D_u8ResrvdSigForCCM2]
  TmSwArch/40 -> [sTmOut_D_u16ResrvdSigForCCM3]
  TmSwArch/41 -> [sTmOut_D_u16ResrvdSigForCCM4]
  TmSwArch/42 -> [sTmOut_Te_s32CooltTSigForDtElec]
  TmSwArch/43 -> [sTmOut_Z_s32CooltFlowForDtElec]
  TmSwArch/44 -> [sTmOut_md_s32HvBattFlwEstmd]
  TmSwArch/45 -> [sTmOut_D_u8HvBattThermReqFb]
  TmSwArch/46 -> [sTmOut_Te_s32AirTFromHeatgEstimd]
  TmSwArch/47 -> [sTmOut_D_u8HpcHpModReq]
  TmSwArch/48 -> [sTmOut_Te_s32ChillerOutT]
  TmSwArch/49 -> [sTmOut_Te_s32CmprDischrgT]
  TmSwArch/50 -> [sTmOut_Te_s32AcCondOutT]
  TmSwArch/51 -> [sTmOut_Te_s32EvapOutT]
  TmSwArch/52 -> [sTmOut_Te_s32InrCondOutT]
  TmSwArch/53 -> [sTmOut_p_s32AcLoSideP]
  TmSwArch/54 -> [sTmOut_D_u8HpcThmMngtSts]
  TmSwArch/55 -> [sTmOut_X_s32HeatrPmpPwmReq]
  TmSwArch/56 -> [sTmOut_Pw_s32HvBattThermPwrCns]
  TmSwArch/57 -> [sTmOut_Pw_s32HvCabinThermPwrCns]
  TmSwArch/58 -> [sTmOut_D_u8BattCooltIndcnReq]
  TmSwArch/59 -> [sTmOut_D_u8EmCooltIndcnReq]
  TmSwArch/60 -> [sTmOut_X_s32FanPwmReq]
  TmSwArch/61 -> [yTmOut_B_PtCoolgPostRunActv]
  TmSwArch/62 -> [sTmOut_D_u8FrntHeatModEnad]
  TmSwArch/63 -> [sTmOut_Pw_s32FrntHeatPwrAllwd]
  TmSwArch/64 -> [yTmOut_B_HpmSov1ActvCmd]
  TmSwArch/65 -> [yTmOut_B_HpmSov2ActvCmd]
  TmSwArch/66 -> [yTmOut_B_HpmSov3ActvCmd]
  TmSwArch/67 -> [sTmOut_X_s32BattCooltPmpReq]
  TmSwArch/68 -> [sTmOut_X_s32EmCooltPmpReq]
  TmSwArch/69 -> [yTmOut_B_ChillerValveReq]
  TmSwArch/70 -> [yTmOut_B_EvaprVlvReqFrnt]
  TmSwArch/71 -> [yTmOut_B_ShttrNetReq]
  TmSwArch/72 -> [sTmOut_P_s32HiSideP]
  TmSwArch/73 -> [sTmOut_Pw_s32HvCoolgPwrNormDes]
  TmSwArch/74 -> [sTmOut_Te_s32OutrCondOutT]
  TmSwArch/75 -> [sTmOut_P_s32LoSideP]
  TmSwArch/76 -> [sTmOut_Te_s32AcCompInletT]
  TmSwArch/77 -> [sTmOut_P_s32HpAcHiSidePNHP]
  TmSwArch/78 -> [sTmOut_D_u8FanPwm2FEnState]
  TmSwArch/79 -> [sTmOut_D_u8VaneCalEnbl2FEnState]
  TmSwArch/80 -> [sTmOut_D_u8GrlShttrTrqBst2FEnState]
  TmSwArch/81 -> [sTmOut_D_u8VaneCtrlAngle2FEnState]
  TmSwArch/82 -> [sTmOut_D_u8ChillerValve2FEnState]
  TmSwArch/83 -> [sTmOut_D_u8EvaprVlvFrnt2FEnState]
  TmSwArch/84 -> [sTmOut_Z_s32AfPred]
  TmSwArch/85 -> [yTmOut_B_EwpAflFlagCooling]
  TmSwArch/86 -> [sTmOut_Pw_s32HvCoolgPwrEvap]
  TmSwArch/87 -> [sTmOut_Pw_s32HvCoolgPwrCns]
  TmSwArch/88 -> [sTmOut_Pw_s32HvCoolgPwrCritDes]
  TmSwArch/89 -> [sTmOut_Pw_s32HvHeatgPwrCritDes]
  TmSwArch/90 -> [sTmOut_Pw_s32HvHeatgPwrNormDes]
  TmSwArch/91 -> [yTmOut_B_CabinCoolingReq]
  TmSwArch/92 -> [yTmOut_B_CabinHeatingReq]
  TmSwArch/93 -> [sTmOut_Pw_s32HvClimaCoolgPwrCritDes]
  TmSwArch/94 -> [sTmOut_Pw_s32HvClimaHeatgPwrCritDes]
  TmSwArch/95 -> [yTmOut_B_HpmSov4ActvCmd]
  TmSwArch/96 -> [yTmOut_B_HpmSov5ActvCmd]
  TmSwArch/97 -> [yTmOut_B_CpsrReqClim]
  TmSwArch/98 -> [sTmOut_Pw_s32HvHeatrPwrCns]
  TmSwArch/99 -> [sTmOut_D_u8HpcCoolgForHvBattSts]
  TmSwArch/100 -> [sTmOut_D_u8SoftwareVersion]
  TmSwArch/101 -> [sTmOut_D_u8CalibrationVersion]
  TmSwArch/102 -> [sTmOut_D_u8HpmSov1Actv2FEnState]
  TmSwArch/103 -> [sTmOut_D_u8HpmSov2Actv2FEnState]
  TmSwArch/104 -> [sTmOut_D_u8HpmSov3Actv2FEnState]
  TmSwArch/105 -> [sTmOut_D_u8PTCPumpSpd2FEnState]
  TmSwArch/106 -> [sTmOut_D_u8EmCooltPmp2FEnState]
  TmSwArch/107 -> [sTmOut_D_u8BattCooltPmp2FEnState]
  TmSwArch/108 -> [sTmOut_D_u8BexvPosnReq2FEnaState]
  TmSwArch/109 -> [sTmOut_D_u8BexvCal2FEnaState]
  TmSwArch/110 -> [sTmOut_D_u8BexvMoveEna2FEnaState]
  TmSwArch/111 -> [sTmOut_D_u8CexvPosnReq2FEnaState]
  TmSwArch/112 -> [sTmOut_D_u8CexvCal2FEnaState]
  TmSwArch/113 -> [sTmOut_D_u8CexvMoveEna2FEnaState]
  TmSwArch/114 -> [sTmOut_D_u8EexvPosnReq2FEnaState]
  TmSwArch/115 -> [sTmOut_D_u8EexvCal2FEnaState]
  TmSwArch/116 -> [sTmOut_D_u8EexvMoveEna2FEnaState]
  TmSwArch/117 -> [sTmOut_D_u8CmprPwrEna2FEnaState]
  TmSwArch/118 -> [sTmOut_D_u8CmprStsEna2FEnaState]
  TmSwArch/119 -> [sTmOut_D_u8CmprSpdEna2FEnaState]
  TmSwArch/120 -> [sTmOut_D_u8PtcPwr2FEnaState]
  TmSwArch/121 -> [sTmOut_D_u8PtcT2FEnaState]
  TmSwArch/122 -> [sTmOut_D_u8PtcEna2FEnaState]
  TmSwArch/123 -> [sTmOut_D_u8BctvVlvPos2FEnaState]
  TmSwArch/124 -> [sTmOut_D_u8BctvVlvRef2FEnaState]
  TmSwArch/125 -> [sTmOut_D_u8BcfvVlvPos2FEnaState]
  TmSwArch/126 -> [sTmOut_D_u8BcfvVlvRef2FEnaState]
  TmSwArch/127 -> [sTmOut_D_u8EctvVlvPos2FEnaState]
  TmSwArch/128 -> [sTmOut_D_u8EctvVlvMoveEna2FEnaState]
  TmSwArch/129 -> [sTmOut_D_u8PtcFlow2FEnaState]
  TmSwArch/130 -> [sTmOut_D_u8ThermalSystemRedn]
  TmSwArch/131 -> [sTmOut_D_u32ThermalSystemFault]
  TmSwArch/132 -> [yTmOut_B_GrlShttrAutoCalibReq]
  TmSwArch/133 -> [sTmOut_Pw_s32RearHeatPwrAllwd]
  TmSwArch/134 -> [sTmOut_D_u8RearHeatModEnad]
  TmSwArch/135 -> [sTmOut_fq_s32PTCPumpPwmFrq]
  TmSwArch/136 -> [sTmOut_fq_s32BattCooltPmpPwmFrq]
  TmSwArch/137 -> [sTmOut_fq_s32EmCooltPmpPwmFrq]
  TmSwArch/138 -> [sTmOut_fq_s32FanPwmFrq]
  TmSwArch/139 -> [sTmOut_D_u8HeatPumpConfig]
  TmSwArch/140 -> [sTmOut_D_u8AdcuConfig]
  TmSwArch/141 -> [sTmOut_D_u8ElecDrivelineConfig]
  TmSwArch/142 -> [sTmOut_D_u8RefrigerantConfig]
  TmSwArch/143 -> [sTmOut_D_u8HvBoostModConfig]
  TmSwArch/144 -> [sTmOut_D_u8BctvFltSt]
  TmSwArch/145 -> [sTmOut_D_u8BcfvFltSt]
  TmSwArch/146 -> [sTmOut_D_u8EctvFltSt]
  TmSwArch/147 -> [sTmOut_D_u8BexvFltSt]
  TmSwArch/148 -> [sTmOut_D_u8CexvFltSt]
  TmSwArch/149 -> [sTmOut_D_u8EexvFltSt]
  TmSwArch/150 -> [sTmOut_D_u8Sov1FltSt]
  TmSwArch/151 -> [sTmOut_D_u8Sov2FltSt]
  TmSwArch/152 -> [sTmOut_D_u8Sov3FltSt]
  TmSwArch/153 -> [sTmOut_D_u8Sov4FltSt]
  TmSwArch/154 -> [sTmOut_D_u8Sov5FltSt]
  TmSwArch/155 -> [sTmOut_D_u8AccmFltSt]
  TmSwArch/156 -> [sTmOut_D_u8HvchFltSt]
  TmSwArch/157 -> [sTmOut_D_u8AgmFltSt]
  TmSwArch/158 -> [yTmOut_B_CarConfigInvalid]
  TmSwArch/159 -> [sTmOut_D_u8HmPmpFltSt]
  TmSwArch/160 -> [sTmOut_D_u8BattPmpFltSt]
  TmSwArch/161 -> [sTmOut_D_u8EmPmpFltSt]
  TmSwArch/162 -> [sTmOut_D_u8FanFltSt]
  TmSwArch/163 -> [sTmOut_D_u8HiSidePNHPFltSt]
  TmSwArch/164 -> [sTmOut_D_u8HiSidePFltSt]
  TmSwArch/165 -> [sTmOut_D_u8LoSidePFltSt]
  TmSwArch/166 -> [sTmOut_D_u8BattClntLvlFltSt]
  TmSwArch/167 -> [sTmOut_D_u8TeEvapFltSt]
  TmSwArch/168 -> [sTmOut_D_u8HvacHexAirTFltSt]
  TmSwArch/169 -> [sTmOut_D_u8HvBattCooltTFltSt]
  TmSwArch/170 -> [sTmOut_D_u8OutrCondOutTFltSt]
  TmSwArch/171 -> [sTmOut_D_u8CmprDischrgTFltSt]
  TmSwArch/172 -> [sTmOut_D_u8EvapOutTFltSt]
  TmSwArch/173 -> [sTmOut_D_u8ChillerOutTFltSt]
  TmSwArch/174 -> [sTmOut_D_u8InrCondOutTFltSt]
  TmSwArch/175 -> [sTmOut_D_u8ClntTforEmCircFltSt]
  TmSwArch/176 -> [sTmOut_D_u8WSMCurMode]
  TmSwArch/177 -> [sTmOut_D_u8HpModeCmd]
  TmSwArch/178 -> [sTmOut_D_u8HpModeMainState]
  TmSwArch/179 -> [sTmOut_D_u8VcEvLowSidePSnrOP]
  TmSwArch/180 -> [sTmOut_D_u8VcEvLowSidePSnrSB]
  TmSwArch/181 -> [sTmOut_D_u8VcEvHiSidePSnrOP]
  TmSwArch/182 -> [sTmOut_D_u8VcEvHiSidePSnrSB]
  TmSwArch/183 -> [sTmOut_D_u8VcEvHiSideTmpSnrSG]
  TmSwArch/184 -> [sTmOut_D_u8VcEvHiSideTmpSnrOP]
  TmSwArch/185 -> [sTmOut_D_u8VcEvChillerOutTSG]
  TmSwArch/186 -> [sTmOut_D_u8VcEvChillerOutTOP]
  TmSwArch/187 -> [sTmOut_D_u8VcEvInrCondOutTSG]
  TmSwArch/188 -> [sTmOut_D_u8VcEvInrCondOutTOP]
  TmSwArch/189 -> [sTmOut_D_u8VcEvEvapOutTSG]
  TmSwArch/190 -> [sTmOut_D_u8VcEvEvapOutTOP]
  TmSwArch/191 -> [sTmOut_D_u8VcEvCmprDischrgTSG]
  TmSwArch/192 -> [sTmOut_D_u8VcEvCmprDischrgTOP]
  TmSwArch/193 -> [sTmOut_D_u8VcEvClntTforEmCircSG]
  TmSwArch/194 -> [sTmOut_D_u8VcEvClntTforEmCircOP]
  TmSwArch/195 -> [sTmOut_D_u8VcEvBattCooltLvlLo]
  TmSwArch/196 -> [sTmOut_D_u8VcEvNoHpHighSidePSnrOP]
  TmSwArch/197 -> [sTmOut_D_u8VcEvNoHpHighSidePSnrSB]
  TmSwArch/198 -> [sTmOut_D_u8VcEvSov1SB]
  TmSwArch/199 -> [sTmOut_D_u8VcEvSov1OP]
  TmSwArch/200 -> [sTmOut_D_u8VcEvSov1SG]
  TmSwArch/201 -> [sTmOut_D_u8VcEvSov2SB]
  TmSwArch/202 -> [sTmOut_D_u8VcEvSov2OP]
  TmSwArch/203 -> [sTmOut_D_u8VcEvSov2SG]
  TmSwArch/204 -> [sTmOut_D_u8VcEvSov3SB]
  TmSwArch/205 -> [sTmOut_D_u8VcEvSov3OP]
  TmSwArch/206 -> [sTmOut_D_u8VcEvSov3SG]
  TmSwArch/207 -> [sTmOut_D_u8VcEvSov4SB]
  TmSwArch/208 -> [sTmOut_D_u8VcEvSov4OP]
  TmSwArch/209 -> [sTmOut_D_u8VcEvSov4SG]
  TmSwArch/210 -> [sTmOut_D_u8VcEvSov5SB]
  TmSwArch/211 -> [sTmOut_D_u8VcEvSov5OP]
  TmSwArch/212 -> [sTmOut_D_u8VcEvSov5SG]
  TmSwArch/213 -> [sTmOut_D_u8VcEvSBFan]
  TmSwArch/214 -> [sTmOut_D_u8VcEvOPFan]
  TmSwArch/215 -> [sTmOut_D_u8VcEvSGFan]
  TmSwArch/216 -> [sTmOut_D_u8VcEvFanOvrTShDwn]
  TmSwArch/217 -> [sTmOut_D_u8VcEvVolErrFan]
  TmSwArch/218 -> [sTmOut_D_u8VcEvBlokFan]
  TmSwArch/219 -> [sTmOut_D_u8VcEvCircutInteFlt]
  TmSwArch/220 -> [sTmOut_D_u8VcEvHmPumpSB]
  TmSwArch/221 -> [sTmOut_D_u8VcEvHmPumpOC]
  TmSwArch/222 -> [sTmOut_D_u8VcEvHmPumpSG]
  TmSwArch/223 -> [sTmOut_D_u8VcEvHmPmpOvrTShutDwn]
  TmSwArch/224 -> [sTmOut_D_u8VcEvHmPmpVolErr]
  TmSwArch/225 -> [sTmOut_D_u8VcEvHmPmpStall]
  TmSwArch/226 -> [sTmOut_D_u8VcEvHmPmpDyRn]
  TmSwArch/227 -> [sTmOut_D_u8VcEvSBBatteryPmp]
  TmSwArch/228 -> [sTmOut_D_u8VcEvOCBatteryPmp]
  TmSwArch/229 -> [sTmOut_D_u8VcEvSGBatteryPmp]
  TmSwArch/230 -> [sTmOut_D_u8VcEvBattPmpOvrTShutDwn]
  TmSwArch/231 -> [sTmOut_D_u8VcEvBattPmpVolErr]
  TmSwArch/232 -> [sTmOut_D_u8VcEvBattPmpStall]
  TmSwArch/233 -> [sTmOut_D_u8VcEvBattPmpDyn]
  TmSwArch/234 -> [sTmOut_D_u8VcEvSBEmotor]
  TmSwArch/235 -> [sTmOut_D_u8VcEvOCEmotor]
  TmSwArch/236 -> [sTmOut_D_u8VcEvSGEmotor]
  TmSwArch/237 -> [sTmOut_D_u8VcEvEmPmpOvrTShutDwn]
  TmSwArch/238 -> [sTmOut_D_u8VcEvEmPmpVolErr]
  TmSwArch/239 -> [sTmOut_D_u8VcEvEmPmpStall]
  TmSwArch/240 -> [sTmOut_D_u8VcEvEmPmpDyRn]
  TmSwArch/241 -> [sTmOut_D_u8VcEvFltTemBCTV]
  TmSwArch/242 -> [sTmOut_D_u8VcEvFltVolBCTV]
  TmSwArch/243 -> [sTmOut_D_u8VcEvBctvIniFail]
  TmSwArch/244 -> [sTmOut_D_u8VcEvBctvBlk]
  TmSwArch/245 -> [sTmOut_D_u8VcEvBctvOthrErr]
  TmSwArch/246 -> [sTmOut_D_u8VcEvBctvNVMFlt]
  TmSwArch/247 -> [sTmOut_D_u8VcEvFltTempBCFV]
  TmSwArch/248 -> [sTmOut_D_u8VcEvFltVolBCFV]
  TmSwArch/249 -> [sTmOut_D_u8VcEvBcfvIniFail]
  TmSwArch/250 -> [sTmOut_D_u8VcEvBcfvBlk]
  TmSwArch/251 -> [sTmOut_D_u8VcEvBcfvOthrErr]
  TmSwArch/252 -> [sTmOut_D_u8VcEvBcfvNVMFlt]
  TmSwArch/253 -> [sTmOut_D_u8VcEvWarnECRV]
  TmSwArch/254 -> [sTmOut_D_u8VcEvFltVolECRV]
  TmSwArch/255 -> [sTmOut_D_u8VcEvEctvDrvMotorFlt]
  TmSwArch/256 -> [sTmOut_D_u8VcEvBexvOvrTempErr]
  TmSwArch/257 -> [sTmOut_D_u8VcEvBexvVoltgRangErr]
  TmSwArch/258 -> [sTmOut_D_u8VcEvBexvIniFail]
  TmSwArch/259 -> [sTmOut_D_u8VcEvBexvBlkErr]
  TmSwArch/260 -> [sTmOut_D_u8VcEvBexvNVMFlt]
  TmSwArch/261 -> [sTmOut_D_u8VcEvCexvOvrTempErr]
  TmSwArch/262 -> [sTmOut_D_u8VcEvCexvVoltgRangErr]
  TmSwArch/263 -> [sTmOut_D_u8VcEvCexvIniFail]
  TmSwArch/264 -> [sTmOut_D_u8VcEvCexvBlkErr]
  TmSwArch/265 -> [sTmOut_D_u8VcEvCexvNVMFlt]
  TmSwArch/266 -> [sTmOut_D_u8VcEvEexvOvrTempErr]
  TmSwArch/267 -> [sTmOut_D_u8VcEvEexvVoltgRangErr]
  TmSwArch/268 -> [sTmOut_D_u8VcEvEexvIniFail]
  TmSwArch/269 -> [sTmOut_D_u8VcEvEexvBlkErr]
  TmSwArch/270 -> [sTmOut_D_u8VcEvEexvNVMFlt]
  TmSwArch/271 -> [sTmOut_D_u8VcEvAccmUSplyErr]
  TmSwArch/272 -> [sTmOut_D_u8VcEvOCACCM]
  TmSwArch/273 -> [sTmOut_D_u8VcEvOPACCM]
  TmSwArch/274 -> [sTmOut_D_u8VcEvCurMotACCM]
  TmSwArch/275 -> [sTmOut_D_u8VcEvCurDrCirtACCM]
  TmSwArch/276 -> [sTmOut_D_u8VcEvRotorLockACCM]
  TmSwArch/277 -> [sTmOut_D_u8VcEvLiquidSluggingACCM]
  TmSwArch/278 -> [sTmOut_D_u8VcEvMemFltAccm]
  TmSwArch/279 -> [sTmOut_D_u8VcEvTM_AGM_OVRTEMP]
  TmSwArch/280 -> [sTmOut_D_u8VcEvAgsVoltErr]
  TmSwArch/281 -> [sTmOut_D_u8VcEvAgsMechErr]
  TmSwArch/282 -> [sTmOut_D_u8VcEvAgsBlk]
  TmSwArch/283 -> [sTmOut_D_u8VcEvAgsElecErr]
  TmSwArch/284 -> [sTmOut_D_u8VcEvAgsNVMFlt]
  TmSwArch/285 -> [sTmOut_D_u8VcEvTempSerIntHVCH]
  TmSwArch/286 -> [sTmOut_D_u8VcEvTempSerOutHVCH]
  TmSwArch/287 -> [sTmOut_D_u8VcEvInterSerTempHVCH]
  TmSwArch/288 -> [sTmOut_D_u8VcEvOvrTempHVCH]
  TmSwArch/289 -> [sTmOut_D_u8VcEvCoolTempOutOfRng]
  TmSwArch/290 -> [sTmOut_D_u8VcEvHWProtHVCH]
  TmSwArch/291 -> [sTmOut_D_u8VcEvIGBTSpOrOpHVCH]
  TmSwArch/292 -> [sTmOut_D_u8VcEvLoVoOvrHVCH]
  TmSwArch/293 -> [sTmOut_D_u8VcEvHiVoOvrHVCH]
  TmSwArch/294 -> [sTmOut_D_u8VcEvCurrOutOfRng]
  TmSwArch/295 -> [sTmOut_D_u8VcEvVolMemErrHVCH]
  TmSwArch/296 -> [sTmOut_D_u8LackRefrigerant]
  TmSwArch/297 -> [sTmOut_D_u8HpcDeiceReq]
  TmSwArch/298 -> [yTmOut_B_HvWtrHeatrActDischrgReq]
  TmSwArch/299 -> [sTmOut_Pw_u32HvEDActHeatgPwrNormDes]
  TmSwArch/300 -> [sTmOut_Pw_u32HvEDActHeatgPwrSumCns]
  TmSwArch/301 -> [sTmOut_D_u8GrlShttrAutoCalibReq2FEnState]
  TmSwArch/302 -> [sTmOut_D_u16ElecDrvHeatgPwrAllwdEEM]
  TmSwArch/303 -> [sTmOut_D_u16HvCoolgPwrAllwdEEM]
  TmSwArch/304 -> [sTmOut_D_u16HvHeatgPwrAllwdEEM]
  TmSwArch/305 -> [sTmOut_D_u8VcEvOVACCM]
  TmSwArch/306 -> [sTmOut_D_u8VcEvAccmIgbtOvrTErr]
  TmSwArch/307 -> [sTmOut_D_u8VcEvAccmSnsrFlt]
  TmSwArch/308 -> [sTmOut_D_u8VcEvAccmPhaseFail]
  TmSwArch/309 -> [sTmOut_D_u8VcEvEctvBlk]
  TmSwArch/310 -> [yTmOut_B_RefLoss]
  TmSwArch/311 -> [sTmOut_n_s32ElacCmprActl]
  TmSwArch/312 -> [sTmOut_Te_s32WtrTInIntk]
  TmSwArch/313 -> [sTmOut_Te_s32WtrTInOutl]
  TmSwArch/314 -> [sTmOut_D_u8VcEvAccmComFlt]
  TmSwArch/315 -> [sTmOut_D_u8VcEvComFltHVCH]
  TmSwArch/316 -> [sTmOut_Z_s32EmCircClntFlwReq]
  TmSwArch/317 -> [sTmOut_Te_s32ChillerOutCooltT]
  TmSwArch/318 -> [sTmOut_D_u8PTCOffState]
  TmSwArch/319 -> [sTmOut_t_s32FanOutSGTLow]
  TmSwArch/320 -> [sTmOut_t_s32BattPmpSGTLow]
  TmSwArch/321 -> [sTmOut_t_s32EmotPmpSGTLow]
  TmSwArch/322 -> [sTmOut_t_s32HmPumpSGTLow]
  TmSwArch/323 -> [sTmOut_D_u8ACOffState]
  TmSwArch/324 -> [sTmOut_D_u8RefriMoreOrLessFltSt]
  TmSwArch/325 -> [sTmOut_Z_u8SystemCurrCOP]
  TmSwArch/326 -> [sTmOut_Z_u8CmpPerfmaCOP]
  [sTmOut_n_u16ElacCmprReq] -> Terminator/1
  [sTmOut_D_u8ElacCmprRelease] -> Terminator1/1
  [yTmOut_B_CexvPosnCalibReq] -> Terminator2/1
  [sTmOut_D_u8CalibrationVersion] -> Terminator3/1
  [sTmOut_D_u8HpmSov1Actv2FEnState] -> Terminator4/1
  [sTmOut_D_u8HpmSov2Actv2FEnState] -> Terminator5/1
  [sTmOut_D_u8HpmSov3Actv2FEnState] -> Terminator6/1
  [sTmOut_D_u8PTCPumpSpd2FEnState] -> Terminator7/1
  [sTmOut_D_u8EmCooltPmp2FEnState] -> Terminator8/1
  [sTmOut_D_u8BattCooltPmp2FEnState] -> Terminator9/1
  [sTmOut_D_u8BexvPosnReq2FEnaState] -> Terminator10/1
  [sTmOut_D_u8BexvCal2FEnaState] -> Terminator11/1
  [sTmOut_D_u8BexvMoveEna2FEnaState] -> Terminator12/1
  [yTmOut_B_CexvPosnMovEnable] -> Terminator13/1
  [sTmOut_D_u8CexvPosnReq2FEnaState] -> Terminator14/1
  [sTmOut_D_u8CexvCal2FEnaState] -> Terminator15/1
  [sTmOut_D_u8CexvMoveEna2FEnaState] -> Terminator16/1
  [sTmOut_D_u8EexvPosnReq2FEnaState] -> Terminator17/1
  [sTmOut_D_u8EexvCal2FEnaState] -> Terminator18/1
  [sTmOut_D_u8EexvMoveEna2FEnaState] -> Terminator19/1
  [sTmOut_D_u8CmprPwrEna2FEnaState] -> Terminator20/1
  [sTmOut_D_u8CmprStsEna2FEnaState] -> Terminator21/1
  [sTmOut_D_u8CmprSpdEna2FEnaState] -> Terminator22/1
  [sTmOut_D_u8PtcPwr2FEnaState] -> Terminator23/1
  [sTmOut_D_u8BctvVlvRefDrvReq] -> Terminator24/1
  [sTmOut_D_u8PtcT2FEnaState] -> Terminator25/1
  [sTmOut_D_u8PtcEna2FEnaState] -> Terminator26/1
  [sTmOut_D_u8BctvVlvPos2FEnaState] -> Terminator27/1
  [sTmOut_D_u8BctvVlvRef2FEnaState] -> Terminator28/1
  [sTmOut_D_u8BcfvVlvPos2FEnaState] -> Terminator29/1
  [sTmOut_D_u8BcfvVlvRef2FEnaState] -> Terminator30/1
  [sTmOut_D_u8EctvVlvPos2FEnaState] -> Terminator31/1
  [sTmOut_D_u8EctvVlvMoveEna2FEnaState] -> Terminator32/1
  [sTmOut_D_u8PtcFlow2FEnaState] -> Terminator33/1
  [sTmOut_D_u8ThermalSystemRedn] -> Terminator34/1
  [sTmOut_X_u8BctvVlvPosReq] -> Terminator35/1
  [sTmOut_D_u32ThermalSystemFault] -> Terminator36/1
  [yTmOut_B_GrlShttrAutoCalibReq] -> Terminator37/1
  [sTmOut_Pw_s32RearHeatPwrAllwd] -> Terminator38/1
  [sTmOut_D_u8RearHeatModEnad] -> Terminator39/1
  [sTmOut_fq_s32PTCPumpPwmFrq] -> Terminator40/1
  [sTmOut_fq_s32BattCooltPmpPwmFrq] -> Terminator41/1
  [sTmOut_fq_s32EmCooltPmpPwmFrq] -> Terminator42/1
  [sTmOut_fq_s32FanPwmFrq] -> Terminator43/1
  [sTmOut_D_u8HeatPumpConfig] -> Terminator44/1
  [sTmOut_D_u8AdcuConfig] -> Terminator45/1
  [sTmOut_D_u8BcfvVlvRefDrvReq] -> Terminator46/1
  [sTmOut_D_u8ElecDrivelineConfig] -> Terminator47/1
  [sTmOut_D_u8RefrigerantConfig] -> Terminator48/1
  [sTmOut_D_u8HvBoostModConfig] -> Terminator49/1
  [sTmOut_D_u8BctvFltSt] -> Terminator50/1
  [sTmOut_D_u8BcfvFltSt] -> Terminator51/1
  [sTmOut_D_u8EctvFltSt] -> Terminator52/1
  [sTmOut_D_u8BexvFltSt] -> Terminator53/1
  [sTmOut_D_u8CexvFltSt] -> Terminator54/1
  [sTmOut_D_u8EexvFltSt] -> Terminator55/1
  [sTmOut_D_u8Sov1FltSt] -> Terminator56/1
  [sTmOut_X_u8BcfvVlvPosReq] -> Terminator57/1
  [sTmOut_D_u8Sov2FltSt] -> Terminator58/1
  [sTmOut_D_u8Sov3FltSt] -> Terminator59/1
  [sTmOut_D_u8Sov4FltSt] -> Terminator60/1
  [sTmOut_D_u8Sov5FltSt] -> Terminator61/1
  [sTmOut_D_u8AccmFltSt] -> Terminator62/1
  [sTmOut_D_u8HvchFltSt] -> Terminator63/1
  [sTmOut_D_u8AgmFltSt] -> Terminator64/1
  [yTmOut_B_CarConfigInvalid] -> Terminator65/1
  [sTmOut_D_u8HmPmpFltSt] -> Terminator66/1
  [sTmOut_D_u8BattPmpFltSt] -> Terminator67/1
  [yTmOut_B_EctvVlvMovEna] -> Terminator68/1
  [sTmOut_D_u8EmPmpFltSt] -> Terminator69/1
  [sTmOut_D_u8FanFltSt] -> Terminator70/1
  [sTmOut_D_u8HiSidePNHPFltSt] -> Terminator71/1
  [sTmOut_D_u8HiSidePFltSt] -> Terminator72/1
  [sTmOut_D_u8LoSidePFltSt] -> Terminator73/1
  [sTmOut_D_u8BattClntLvlFltSt] -> Terminator74/1
  [sTmOut_D_u8TeEvapFltSt] -> Terminator75/1
  [sTmOut_D_u8HvacHexAirTFltSt] -> Terminator76/1
  [sTmOut_D_u8HvBattCooltTFltSt] -> Terminator77/1
  [sTmOut_D_u8OutrCondOutTFltSt] -> Terminator78/1
  [sTmOut_D_u8EctvVlvPosReq] -> Terminator79/1
  [sTmOut_D_u8CmprDischrgTFltSt] -> Terminator80/1
  [sTmOut_D_u8EvapOutTFltSt] -> Terminator81/1
  [sTmOut_D_u8ChillerOutTFltSt] -> Terminator82/1
  [sTmOut_D_u8InrCondOutTFltSt] -> Terminator83/1
  [sTmOut_D_u8ClntTforEmCircFltSt] -> Terminator84/1
  [sTmOut_D_u8WSMCurMode] -> Terminator85/1
  [sTmOut_D_u8HpModeCmd] -> Terminator86/1
  [sTmOut_D_u8HpModeMainState] -> Terminator87/1
  [sTmOut_D_u8VcEvLowSidePSnrOP] -> Terminator88/1
  [sTmOut_D_u8VcEvLowSidePSnrSB] -> Terminator89/1
  [sTmOut_Te_s32PTCTempReq] -> Terminator90/1
  [sTmOut_D_u8VcEvHiSidePSnrOP] -> Terminator91/1
  [sTmOut_D_u8VcEvHiSidePSnrSB] -> Terminator92/1
  [sTmOut_D_u8VcEvHiSideTmpSnrSG] -> Terminator93/1
  [sTmOut_D_u8VcEvHiSideTmpSnrOP] -> Terminator94/1
  [sTmOut_D_u8VcEvChillerOutTSG] -> Terminator95/1
  [sTmOut_D_u8VcEvChillerOutTOP] -> Terminator96/1
  [sTmOut_D_u8VcEvInrCondOutTSG] -> Terminator97/1
  [sTmOut_D_u8VcEvInrCondOutTOP] -> Terminator98/1
  [sTmOut_D_u8VcEvEvapOutTSG] -> Terminator99/1
  [sTmOut_D_u8VcEvEvapOutTOP] -> Terminator100/1
  [sTmOut_Z_s32PTCCoolantFlowrate] -> Terminator101/1
  [sTmOut_D_u8VcEvCmprDischrgTSG] -> Terminator102/1
  [sTmOut_D_u8VcEvCmprDischrgTOP] -> Terminator103/1
  [sTmOut_D_u8VcEvClntTforEmCircSG] -> Terminator104/1
  [sTmOut_D_u8VcEvClntTforEmCircOP] -> Terminator105/1
  [sTmOut_D_u8VcEvBattCooltLvlLo] -> Terminator106/1
  [sTmOut_D_u8VcEvNoHpHighSidePSnrOP] -> Terminator107/1
  [sTmOut_D_u8VcEvNoHpHighSidePSnrSB] -> Terminator108/1
  [sTmOut_D_u8VcEvSov1SB] -> Terminator109/1
  [sTmOut_D_u8VcEvSov1OP] -> Terminator110/1
  [sTmOut_D_u8VcEvSov1SG] -> Terminator111/1
  [sTmOut_Pw_s32ElacCmprMax] -> Terminator112/1
  [sTmOut_Pw_s32PTCPowerAlld] -> Terminator113/1
  [sTmOut_D_u8VcEvSov2SB] -> Terminator114/1
  [sTmOut_D_u8VcEvSov2OP] -> Terminator115/1
  [sTmOut_D_u8VcEvSov2SG] -> Terminator116/1
  [sTmOut_D_u8VcEvSov3SB] -> Terminator117/1
  [sTmOut_D_u8VcEvSov3OP] -> Terminator118/1
  [sTmOut_D_u8VcEvSov3SG] -> Terminator119/1
  [sTmOut_D_u8VcEvSov4SB] -> Terminator120/1
  [sTmOut_D_u8VcEvSov4OP] -> Terminator121/1
  [sTmOut_D_u8VcEvSov4SG] -> Terminator122/1
  [sTmOut_D_u8VcEvSov5SB] -> Terminator123/1
  [yTmOut_B_PTCEnabled] -> Terminator124/1
  [sTmOut_D_u8VcEvSov5OP] -> Terminator125/1
  [sTmOut_D_u8VcEvSov5SG] -> Terminator126/1
  [sTmOut_D_u8VcEvSBFan] -> Terminator127/1
  [sTmOut_D_u8VcEvOPFan] -> Terminator128/1
  [sTmOut_D_u8VcEvSGFan] -> Terminator129/1
  [sTmOut_D_u8VcEvFanOvrTShDwn] -> Terminator130/1
  [sTmOut_D_u8VcEvVolErrFan] -> Terminator131/1
  [sTmOut_D_u8VcEvBlokFan] -> Terminator132/1
  [sTmOut_D_u8VcEvCircutInteFlt] -> Terminator133/1
  [sTmOut_D_u8VcEvHmPumpSB] -> Terminator134/1
  [yTmOut_B_VaneCalEnbl] -> Terminator135/1
  [sTmOut_D_u8VcEvHmPumpOC] -> Terminator136/1
  [sTmOut_D_u8VcEvHmPumpSG] -> Terminator137/1
  [sTmOut_D_u8VcEvHmPmpOvrTShutDwn] -> Terminator138/1
  [sTmOut_D_u8VcEvHmPmpVolErr] -> Terminator139/1
  [sTmOut_D_u8VcEvHmPmpStall] -> Terminator140/1
  [sTmOut_D_u8VcEvHmPmpDyRn] -> Terminator141/1
  [sTmOut_D_u8VcEvSBBatteryPmp] -> Terminator142/1
  [sTmOut_D_u8VcEvOCBatteryPmp] -> Terminator143/1
  [sTmOut_D_u8VcEvSGBatteryPmp] -> Terminator144/1
  [sTmOut_D_u8VcEvBattPmpOvrTShutDwn] -> Terminator145/1
  [sTmOut_Z_s32VaneCtrlAngleReq] -> Terminator146/1
  [sTmOut_D_u8VcEvBattPmpVolErr] -> Terminator147/1
  [sTmOut_D_u8VcEvBattPmpStall] -> Terminator148/1
  [sTmOut_D_u8VcEvBattPmpDyn] -> Terminator149/1
  [sTmOut_D_u8VcEvSBEmotor] -> Terminator150/1
  [sTmOut_D_u8VcEvOCEmotor] -> Terminator151/1
  [sTmOut_D_u8VcEvSGEmotor] -> Terminator152/1
  [sTmOut_D_u8VcEvEmPmpOvrTShutDwn] -> Terminator153/1
  [sTmOut_D_u8VcEvEmPmpVolErr] -> Terminator154/1
  [sTmOut_D_u8VcEvEmPmpStall] -> Terminator155/1
  [sTmOut_D_u8VcEvEmPmpDyRn] -> Terminator156/1
  [sTmOut_D_u8GrlShttrTrqBstReq] -> Terminator157/1
  [sTmOut_D_u8VcEvFltTemBCTV] -> Terminator158/1
  [sTmOut_D_u8VcEvFltVolBCTV] -> Terminator159/1
  [sTmOut_D_u8VcEvBctvIniFail] -> Terminator160/1
  [sTmOut_D_u8VcEvBctvBlk] -> Terminator161/1
  [sTmOut_D_u8VcEvBctvOthrErr] -> Terminator162/1
  [sTmOut_D_u8VcEvBctvNVMFlt] -> Terminator163/1
  [sTmOut_D_u8VcEvFltTempBCFV] -> Terminator164/1
  [sTmOut_D_u8VcEvFltVolBCFV] -> Terminator165/1
  [sTmOut_D_u8VcEvBcfvIniFail] -> Terminator166/1
  [sTmOut_D_u8VcEvBcfvBlk] -> Terminator167/1
  [sTmOut_D_u8Sov1OnOffSts] -> Terminator168/1
  [sTmOut_D_u8VcEvBcfvOthrErr] -> Terminator169/1
  [sTmOut_D_u8VcEvBcfvNVMFlt] -> Terminator170/1
  [sTmOut_D_u8VcEvWarnECRV] -> Terminator171/1
  [sTmOut_D_u8VcEvFltVolECRV] -> Terminator172/1
  [sTmOut_D_u8VcEvEctvDrvMotorFlt] -> Terminator173/1
  [sTmOut_D_u8VcEvBexvOvrTempErr] -> Terminator174/1
  [sTmOut_D_u8VcEvBexvVoltgRangErr] -> Terminator175/1
  [sTmOut_D_u8VcEvBexvIniFail] -> Terminator176/1
  [sTmOut_D_u8VcEvBexvBlkErr] -> Terminator177/1
  [sTmOut_D_u8VcEvBexvNVMFlt] -> Terminator178/1
  [sTmOut_D_u8Sov2OnOffSts] -> Terminator179/1
  [sTmOut_D_u8VcEvCexvOvrTempErr] -> Terminator180/1
  [sTmOut_D_u8VcEvCexvVoltgRangErr] -> Terminator181/1
  [sTmOut_D_u8VcEvCexvIniFail] -> Terminator182/1
  [sTmOut_D_u8VcEvCexvBlkErr] -> Terminator183/1
  [sTmOut_D_u8VcEvCexvNVMFlt] -> Terminator184/1
  [sTmOut_D_u8VcEvEexvOvrTempErr] -> Terminator185/1
  [sTmOut_D_u8VcEvEexvVoltgRangErr] -> Terminator186/1
  [sTmOut_D_u8VcEvEexvIniFail] -> Terminator187/1
  [sTmOut_D_u8VcEvEexvBlkErr] -> Terminator188/1
  [sTmOut_D_u8VcEvEexvNVMFlt] -> Terminator189/1
  [sTmOut_D_u8AirCondCmpsrStats] -> Terminator190/1
  [sTmOut_D_u8VcEvAccmUSplyErr] -> Terminator191/1
  [sTmOut_D_u8VcEvOCACCM] -> Terminator192/1
  [sTmOut_D_u8VcEvOPACCM] -> Terminator193/1
  [sTmOut_D_u8VcEvCurMotACCM] -> Terminator194/1
  [sTmOut_D_u8VcEvCurDrCirtACCM] -> Terminator195/1
  [sTmOut_D_u8VcEvRotorLockACCM] -> Terminator196/1
  [sTmOut_D_u8VcEvLiquidSluggingACCM] -> Terminator197/1
  [sTmOut_D_u8VcEvMemFltAccm] -> Terminator198/1
  [sTmOut_D_u8VcEvTM_AGM_OVRTEMP] -> Terminator199/1
  [sTmOut_D_u8VcEvAgsVoltErr] -> Terminator200/1
  [sTmOut_t_u32CmprRunTime] -> Terminator201/1
  [sTmOut_D_u8VcEvAgsMechErr] -> Terminator202/1
  [sTmOut_D_u8VcEvAgsBlk] -> Terminator203/1
  [sTmOut_D_u8VcEvAgsElecErr] -> Terminator204/1
  [sTmOut_D_u8VcEvAgsNVMFlt] -> Terminator205/1
  [sTmOut_D_u8VcEvTempSerIntHVCH] -> Terminator206/1
  [sTmOut_D_u8VcEvTempSerOutHVCH] -> Terminator207/1
  [sTmOut_D_u8VcEvInterSerTempHVCH] -> Terminator208/1
  [sTmOut_D_u8VcEvOvrTempHVCH] -> Terminator209/1
  [sTmOut_D_u8VcEvCoolTempOutOfRng] -> Terminator210/1
  [sTmOut_D_u8VcEvHWProtHVCH] -> Terminator211/1
  [yTmOut_B_CoolgLimd] -> Terminator212/1
  [sTmOut_D_u8VcEvIGBTSpOrOpHVCH] -> Terminator213/1
  [sTmOut_D_u8VcEvLoVoOvrHVCH] -> Terminator214/1
  [sTmOut_D_u8VcEvHiVoOvrHVCH] -> Terminator215/1
  [sTmOut_D_u8VcEvCurrOutOfRng] -> Terminator216/1
  [sTmOut_D_u8VcEvVolMemErrHVCH] -> Terminator217/1
  [sTmOut_D_u8LackRefrigerant] -> Terminator218/1
  [sTmOut_D_u8HpcDeiceReq] -> Terminator219/1
  [yTmOut_B_HvWtrHeatrActDischrgReq] -> Terminator220/1
  [sTmOut_Pw_u32HvEDActHeatgPwrNormDes] -> Terminator221/1
  [sTmOut_Pw_u32HvEDActHeatgPwrSumCns] -> Terminator222/1
  [sTmOut_X_s32EexvVlvPosReq] -> Terminator223/1
  [sTmOut_D_u8CoolgLoad] -> Terminator224/1
  [sTmOut_D_u8GrlShttrAutoCalibReq2FEnState] -> Terminator225/1
  [sTmOut_D_u16ElecDrvHeatgPwrAllwdEEM] -> Terminator226/1
  [sTmOut_D_u16HvCoolgPwrAllwdEEM] -> Terminator227/1
  [sTmOut_D_u16HvHeatgPwrAllwdEEM] -> Terminator228/1
  [sTmOut_D_u8VcEvOVACCM] -> Terminator229/1
  [sTmOut_D_u8VcEvAccmIgbtOvrTErr] -> Terminator230/1
  [sTmOut_D_u8VcEvAccmSnsrFlt] -> Terminator231/1
  [sTmOut_D_u8VcEvAccmPhaseFail] -> Terminator232/1
  [sTmOut_D_u8VcEvEctvBlk] -> Terminator233/1
  [yTmOut_B_RefLoss] -> Terminator234/1
  [sTmOut_X_s32PTCPumpSpdReq] -> Terminator235/1
  [sTmOut_n_s32ElacCmprActl] -> Terminator236/1
  [sTmOut_Te_s32WtrTInIntk] -> Terminator237/1
  [sTmOut_Te_s32WtrTInOutl] -> Terminator238/1
  [sTmOut_D_u8VcEvAccmComFlt] -> Terminator239/1
  [sTmOut_D_u8VcEvComFltHVCH] -> Terminator240/1
  [sTmOut_Z_s32EmCircClntFlwReq] -> Terminator241/1
  [sTmOut_Te_s32ChillerOutCooltT] -> Terminator242/1
  [sTmOut_D_u8PTCOffState] -> Terminator243/1
  [sTmOut_t_s32FanOutSGTLow] -> Terminator244/1
  [sTmOut_t_s32BattPmpSGTLow] -> Terminator245/1
  [sTmOut_Pw_s32HtrPmpPwrCns] -> Terminator246/1
  [sTmOut_t_s32EmotPmpSGTLow] -> Terminator247/1
  [sTmOut_t_s32HmPumpSGTLow] -> Terminator248/1
  [sTmOut_D_u8ACOffState] -> Terminator249/1
  [sTmOut_D_u8RefriMoreOrLessFltSt] -> Terminator250/1
  [sTmOut_Z_u8SystemCurrCOP] -> Terminator251/1
  [sTmOut_Z_u8CmpPerfmaCOP] -> Terminator252/1
  [sTmOut_Pw_s32HvBattPmpPwrCns] -> Terminator253/1
  [sTmOut_Pw_s32EldtPmpPwrCns] -> Terminator254/1
  [sTmOut_n_s32HeatrPmpSpdAct] -> Terminator255/1
  [sTmOut_Pw_s32FanPwrCns] -> Terminator256/1
  [sTmOut_D_u8ResrvdSigForCCM1] -> Terminator257/1
  [sTmOut_D_u8ResrvdSigForCCM2] -> Terminator258/1
  [sTmOut_D_u16ResrvdSigForCCM3] -> Terminator259/1
  [yTmOut_B_EexvPosnCalibReq] -> Terminator260/1
  [sTmOut_D_u16ResrvdSigForCCM4] -> Terminator261/1
  [sTmOut_Te_s32CooltTSigForDtElec] -> Terminator262/1
  [sTmOut_Z_s32CooltFlowForDtElec] -> Terminator263/1
  [sTmOut_md_s32HvBattFlwEstmd] -> Terminator264/1
  [sTmOut_D_u8HvBattThermReqFb] -> Terminator265/1
  [sTmOut_Te_s32AirTFromHeatgEstimd] -> Terminator266/1
  [sTmOut_D_u8HpcHpModReq] -> Terminator267/1
  [sTmOut_Te_s32ChillerOutT] -> Terminator268/1
  [sTmOut_Te_s32CmprDischrgT] -> Terminator269/1
  [sTmOut_Te_s32AcCondOutT] -> Terminator270/1
  [yTmOut_B_EexvPosnMovEnable] -> Terminator271/1
  [sTmOut_Te_s32EvapOutT] -> Terminator272/1
  [sTmOut_Te_s32InrCondOutT] -> Terminator273/1
  [sTmOut_p_s32AcLoSideP] -> Terminator274/1
  [sTmOut_D_u8HpcThmMngtSts] -> Terminator275/1
  [sTmOut_X_s32HeatrPmpPwmReq] -> Terminator276/1
  [sTmOut_Pw_s32HvBattThermPwrCns] -> Terminator277/1
  [sTmOut_Pw_s32HvCabinThermPwrCns] -> Terminator278/1
  [sTmOut_D_u8BattCooltIndcnReq] -> Terminator279/1
  [sTmOut_D_u8EmCooltIndcnReq] -> Terminator280/1
  [sTmOut_X_s32FanPwmReq] -> Terminator281/1
  [sTmOut_X_s32BexvVlvPosReq] -> Terminator282/1
  [yTmOut_B_PtCoolgPostRunActv] -> Terminator283/1
  [sTmOut_D_u8FrntHeatModEnad] -> Terminator284/1
  [sTmOut_Pw_s32FrntHeatPwrAllwd] -> Terminator285/1
  [yTmOut_B_HpmSov1ActvCmd] -> Terminator286/1
  [yTmOut_B_HpmSov2ActvCmd] -> Terminator287/1
  [yTmOut_B_HpmSov3ActvCmd] -> Terminator288/1
  [sTmOut_X_s32BattCooltPmpReq] -> Terminator289/1
  [sTmOut_X_s32EmCooltPmpReq] -> Terminator290/1
  [yTmOut_B_ChillerValveReq] -> Terminator291/1
  [yTmOut_B_EvaprVlvReqFrnt] -> Terminator292/1
  [yTmOut_B_BexvPosnCalibReq] -> Terminator293/1
  [yTmOut_B_ShttrNetReq] -> Terminator294/1
  [sTmOut_P_s32HiSideP] -> Terminator295/1
  [sTmOut_Pw_s32HvCoolgPwrNormDes] -> Terminator296/1
  [sTmOut_Te_s32OutrCondOutT] -> Terminator297/1
  [sTmOut_P_s32LoSideP] -> Terminator298/1
  [sTmOut_Te_s32AcCompInletT] -> Terminator299/1
  [sTmOut_P_s32HpAcHiSidePNHP] -> Terminator300/1
  [sTmOut_D_u8FanPwm2FEnState] -> Terminator301/1
  [sTmOut_D_u8VaneCalEnbl2FEnState] -> Terminator302/1
  [sTmOut_D_u8GrlShttrTrqBst2FEnState] -> Terminator303/1
  [yTmOut_B_BexvPosnMovEnable] -> Terminator304/1
  [sTmOut_D_u8VaneCtrlAngle2FEnState] -> Terminator305/1
  [sTmOut_D_u8ChillerValve2FEnState] -> Terminator306/1
  [sTmOut_D_u8EvaprVlvFrnt2FEnState] -> Terminator307/1
  [sTmOut_Z_s32AfPred] -> Terminator308/1
  [yTmOut_B_EwpAflFlagCooling] -> Terminator309/1
  [sTmOut_Pw_s32HvCoolgPwrEvap] -> Terminator310/1
  [sTmOut_Pw_s32HvCoolgPwrCns] -> Terminator311/1
  [sTmOut_Pw_s32HvCoolgPwrCritDes] -> Terminator312/1
  [sTmOut_Pw_s32HvHeatgPwrCritDes] -> Terminator313/1
  [sTmOut_Pw_s32HvHeatgPwrNormDes] -> Terminator314/1
  [sTmOut_X_s32CexvVlvPosReq] -> Terminator315/1
  [yTmOut_B_CabinCoolingReq] -> Terminator316/1
  [yTmOut_B_CabinHeatingReq] -> Terminator317/1
  [sTmOut_Pw_s32HvClimaCoolgPwrCritDes] -> Terminator318/1
  [sTmOut_Pw_s32HvClimaHeatgPwrCritDes] -> Terminator319/1
  [yTmOut_B_HpmSov4ActvCmd] -> Terminator320/1
  [yTmOut_B_HpmSov5ActvCmd] -> Terminator321/1
  [yTmOut_B_CpsrReqClim] -> Terminator322/1
  [sTmOut_Pw_s32HvHeatrPwrCns] -> Terminator323/1
  [sTmOut_D_u8HpcCoolgForHvBattSts] -> Terminator324/1
  [sTmOut_D_u8SoftwareVersion] -> Terminator325/1
  Ground/1 -> [sTmIn_L_s32WhlMotCooltFlowMinReq]
  Ground1/1 -> [sTmIn_Te_s32WhlMotSysCooltT]
  Ground2/1 -> [sTmIn_D_u8OnBdChrgrHndlSts]
  Ground3/1 -> [yTmIn_B_Sov4OPTF]
  Ground4/1 -> [yTmIn_B_Sov4OPflg]
  Ground5/1 -> [yTmIn_B_Sov4SBTF]
  Ground6/1 -> [yTmIn_B_Sov4SBflg]
  Ground7/1 -> [yTmIn_B_Sov4SGTF]
  Ground8/1 -> [yTmIn_B_Sov4SGflg]
  Ground9/1 -> [yTmIn_B_Sov5OPTF]
  Ground10/1 -> [yTmIn_B_Sov5OPflg]
  Ground11/1 -> [yTmIn_B_Sov5SBTF]
  Ground12/1 -> [yTmIn_B_Sov5SBflg]
  Ground13/1 -> [sTmIn_Te_s32ObcActl]
  Ground14/1 -> [yTmIn_B_Sov5SGTF]
  Ground15/1 -> [yTmIn_B_Sov5SGflg]
  Ground16/1 -> [sTmIn_X_s32BattCooltPmpReq2F]
  Ground17/1 -> [sTmIn_X_s32PTCPumpSpdReq2F]
  Ground18/1 -> [sTmIn_D_u8CmprStsEnaReq2F]
  Ground19/1 -> [sTmIn_n_s32CmprSpdReq2F]
  Ground20/1 -> [sTmIn_Pw_s32CmprPwrEnaReq2F]
  Ground21/1 -> [sTmIn_D_u8GrlShttrTrqBstReq2F]
  Ground22/1 -> [sTmIn_D_u8BcfvVlvRefReq2F]
  Ground23/1 -> [sTmIn_X_u8BcfvVlvPosReq2F]
  Ground24/1 -> [sTmIn_L_s32OnBdChrgrMinCooltFlow]
  Ground25/1 -> [sTmIn_D_u8BctvVlvRefReq2F]
  Ground26/1 -> [sTmIn_X_u8BctvVlvPosReq2F]
  Ground27/1 -> [yTmIn_B_BExvCalReq2F]
  Ground28/1 -> [yTmIn_B_BExvMoveEnReq2F]
  Ground29/1 -> [sTmIn_X_s32BExvPosnReq2F]
  Ground30/1 -> [yTmIn_B_CExvCalReq2F]
  Ground31/1 -> [yTmIn_B_CExvMoveEnaReq2F]
  Ground32/1 -> [sTmIn_X_s32CExvPosnReq2F]
  Ground33/1 -> [yTmIn_B_EctvVlvMoveEnaReq2F]
  Ground34/1 -> [sTmIn_X_u8EctvVlvPosReq2F]
  Ground35/1 -> [sTmIn_Te_s32OnBdChrgrCooltT]
  Ground36/1 -> [yTmIn_B_EExvCalReq2F]
  Ground37/1 -> [yTmIn_B_EExvMoveEnaReq2F]
  Ground38/1 -> [sTmIn_X_s32EExvPosnReq2F]
  Ground39/1 -> [yTmIn_B_PtcEnaReq2F]
  Ground40/1 -> [sTmIn_Pw_s32PtcPwrReq2F]
  Ground41/1 -> [sTmIn_Te_s32PtcTReq2F]
  Ground42/1 -> [sTmIn_L_s32PtcFlowReq2F]
  Ground43/1 -> [sTmIn_X_s32FanPwmReq2F]
  Ground44/1 -> [sTmIn_Z_s32VaneCtrlAngleReq2F]
  Ground45/1 -> [sTmIn_X_s32EmCooltPmpReq2F]
  Ground46/1 -> [sTmIn_Te_s32TDcDcCoolt]
  Ground47/1 -> [yTmIn_B_HpmSov1ActvCmd2F]
  Ground48/1 -> [yTmIn_B_HpmSov2ActvCmd2F]
  Ground49/1 -> [yTmIn_B_HpmSov3ActvCmd2F]
  Ground50/1 -> [yTmIn_B_EvaprVlvReqFrnt2F]
  Ground51/1 -> [yTmIn_B_ChillerValveReq2F]
  Ground52/1 -> [yTmIn_B_VaneCalEnbl2F]
  Ground53/1 -> [yTmIn_B_HpmSov1Actv2FReq]
  Ground54/1 -> [yTmIn_B_HpmSov2Actv2FReq]
  Ground55/1 -> [yTmIn_B_HpmSov3Actv2FReq]
  Ground56/1 -> [yTmIn_B_BattPmp2FReq]
  Ground57/1 -> [sTmIn_D_u8HvBattCooltLvl]
  Ground58/1 -> [yTmIn_B_PTCPumpSpd2FReq]
  Ground59/1 -> [yTmIn_B_EvaprVlvFrnt2FReq]
  Ground60/1 -> [yTmIn_B_CmprPwrEna2FReq]
  Ground61/1 -> [yTmIn_B_CmprSpd2FReq]
  Ground62/1 -> [yTmIn_B_CmprStsEna2FReq]
  Ground63/1 -> [yTmIn_B_GrlShttrTrqBst2FReq]
  Ground64/1 -> [yTmIn_B_BcfvVlvPos2FReq]
  Ground65/1 -> [yTmIn_B_BcfvVlvRef2FReq]
  Ground66/1 -> [yTmIn_B_BctvVlvPos2FReq]
  Ground67/1 -> [yTmIn_B_BctvVlvRef2FReq]
  Ground68/1 -> [sTmIn_D_u8DCChrgnHndlSts]
  Ground69/1 -> [yTmIn_B_BExvCal2FReq]
  Ground70/1 -> [yTmIn_B_BExvMoveEna2FReq]
  Ground71/1 -> [yTmIn_B_BExvPosn2FReq]
  Ground72/1 -> [yTmIn_B_CExvCal2FReq]
  Ground73/1 -> [yTmIn_B_CExvMoveEna2FReq]
  Ground74/1 -> [yTmIn_B_CExvPosn2FReq]
  Ground75/1 -> [yTmIn_B_ChillerValve2FReq]
  Ground76/1 -> [yTmIn_B_EctvVlvMoveEna2FReq]
  Ground77/1 -> [yTmIn_B_EctvVlvPos2FReq]
  Ground78/1 -> [yTmIn_B_EExvCal2FReq]
  Ground79/1 -> [sTmIn_D_u8HvBattCoolgReq]
  Ground80/1 -> [yTmIn_B_EExvMoveEna2FReq]
  Ground81/1 -> [yTmIn_B_EExvPosn2FReq]
  Ground82/1 -> [yTmIn_B_PtcEna2FReq]
  Ground83/1 -> [yTmIn_B_PtcFlow2FReq]
  Ground84/1 -> [yTmIn_B_PtcPwr2FReq]
  Ground85/1 -> [yTmIn_B_PtcT2FReq]
  Ground86/1 -> [yTmIn_B_FanPwm2FReq]
  Ground87/1 -> [yTmIn_B_VaneCalEnbl2FReq]
  Ground88/1 -> [yTmIn_B_VaneCtrlAngle2FReq]
  Ground89/1 -> [yTmIn_B_EmCooltPmp2FReq]
  Ground90/1 -> [sTmIn_D_u8HvBattHeatgReq]
  Ground91/1 -> [sTmIn_D_u8AcCmpr]
  Ground92/1 -> [sTmIn_D_u8BattCoolLelIn]
  Ground93/1 -> [sTmIn_D_u8EldtCoolLelIn]
  Ground94/1 -> [sTmIn_D_u8ForHvacTyp]
  Ground95/1 -> [sTmIn_D_u8HeatPump]
  Ground96/1 -> [sTmIn_D_u8HvacRe]
  Ground97/1 -> [sTmIn_D_u8Refrigerant]
  Ground98/1 -> [sTmIn_D_u8ShutterConfig]
  Ground99/1 -> [sTmIn_U_s32AcCompDischrgT]
  Ground100/1 -> [sTmIn_U_s32AcCompInletT]
  Ground101/1 -> [sTmIn_D_u8HvBattThermReq]
  Ground102/1 -> [sTmIn_U_s32AcCondOutT]
  Ground103/1 -> [sTmIn_U_s32AcEvapOutT]
  Ground104/1 -> [sTmIn_U_s32AcIntelCondOutT]
  Ground105/1 -> [sTmIn_U_s32HiSideP]
  Ground106/1 -> [sTmIn_U_s32HiSidePNHP]
  Ground107/1 -> [sTmIn_U_s32LoSideP]
  Ground108/1 -> [sTmIn_U_s32CooltTSigForDtElec]
  Ground109/1 -> [yTmIn_B_CPSRFbSt]
  Ground110/1 -> [sTmIn_U_s32BattVolt]
  Ground111/1 -> [yTmIn_B_HvBattThermModUD]
  Ground112/1 -> [sTmIn_D_u8EradCoolReq]
  Ground113/1 -> [sTmIn_D_u16HVvBattLimnIndcn]
  Ground114/1 -> [sTmIn_D_u8EexvBlkErr]
  Ground115/1 -> [sTmIn_D_u8EexvElecStsErr]
  Ground116/1 -> [sTmIn_D_u8EexvNVMFlt]
  Ground117/1 -> [sTmIn_D_u8EexvOvrTempErr]
  Ground118/1 -> [sTmIn_D_u8EexvVoltgRangErr]
  Ground119/1 -> [sTmIn_D_u8EexvOvrTrvlErr]
  Ground120/1 -> [sTmIn_D_u8CexvBlkErr]
  Ground121/1 -> [sTmIn_D_u8CexvElecStsErr]
  Ground122/1 -> [sTmIn_D_u8CexvNVMFlt]
  Ground123/1 -> [sTmIn_D_u8CexvOvrTempErr]
  Ground124/1 -> [sTmIn_Pw_s32HvBattClimaPwr]
  Ground125/1 -> [sTmIn_D_u8CexvVoltgRangErr]
  Ground126/1 -> [sTmIn_D_u8CexvOvrTrvlErr]
  Ground127/1 -> [sTmIn_D_u8EctvFaultSts]
  Ground128/1 -> [sTmIn_D_u8EctvTempSts]
  Ground129/1 -> [sTmIn_D_u8EctvVoltSts]
  Ground130/1 -> [sTmIn_D_u8BexvBlkErr]
  Ground131/1 -> [sTmIn_D_u8BexvCalibSts]
  Ground132/1 -> [sTmIn_D_u8BexvElecStsErr]
  Ground133/1 -> [sTmIn_D_u8BexvNVMFlt]
  Ground134/1 -> [sTmIn_D_u8BexvOvrTempErr]
  Ground135/1 -> [sTmIn_Te_s32BattHv]
  Ground136/1 -> [sTmIn_D_u8BexvOvrTrvlErr]
  Ground137/1 -> [sTmIn_D_u8BexvPreHeatgSts]
  Ground138/1 -> [sTmIn_D_u8BexvVoltgRangErr]
  Ground139/1 -> [sTmIn_X_s32BexvPosSts]
  Ground140/1 -> [yTmIn_B_BexvComFault]
  Ground141/1 -> [sTmIn_D_u8BcfvFaultSts]
  Ground142/1 -> [sTmIn_D_u8BcfvNVMFlt]
  Ground143/1 -> [sTmIn_D_u8BcfvTempSts]
  Ground144/1 -> [sTmIn_D_u8BcfvVoltSts]
  Ground145/1 -> [sTmIn_D_u8BctvFaultSts]
  Ground146/1 -> [sTmIn_Te_s32HvBattCooltT]
  Ground147/1 -> [sTmIn_D_u8BctvNVMFlt]
  Ground148/1 -> [sTmIn_D_u8BctvTempSts]
  Ground149/1 -> [sTmIn_D_u8BctvVoltSts]
  Ground150/1 -> [sTmIn_X_s32BctvPosSts]
  Ground151/1 -> [sTmIn_D_u8CmprRAMFault]
  Ground152/1 -> [sTmIn_D_u8CmprROMFault]
  Ground153/1 -> [sTmIn_D_u8CmprRotorLockStat]
  Ground154/1 -> [sTmIn_D_u8CmprSts1]
  Ground155/1 -> [sTmIn_D_u8HVoltResonanceStat]
  Ground156/1 -> [sTmIn_D_u8InCurrOverCurrStat]
  Ground157/1 -> [sTmIn_Te_s32HvBattCooltTReq]
  Ground158/1 -> [sTmIn_D_u8LiquidSluggingStat]
  Ground159/1 -> [sTmIn_D_u8MotorCurrOverCurrStat]
  Ground160/1 -> [sTmIn_D_u8OverMotorCurrStat]
  Ground161/1 -> [sTmIn_D_u8OverPowerStat]
  Ground162/1 -> [sTmIn_I_s32ElacCmprHvActl]
  Ground163/1 -> [sTmIn_n_s32ElacCmprActl]
  Ground164/1 -> [sTmIn_Te_s32CmprT1]
  Ground165/1 -> [sTmIn_U_s32ElacCmprHvActl]
  Ground166/1 -> [sTmIn_D_u8ErrRespAGM]
  Ground167/1 -> [sTmIn_D_u8GrlActTrqBoost]
  Ground168/1 -> [sTmIn_L_s32HvBattCoolFlow1]
  Ground169/1 -> [sTmIn_D_u8GrlHldTrqActive]
  Ground170/1 -> [sTmIn_D_u8GrlShttrMoveActive]
  Ground171/1 -> [sTmIn_D_u8GrlShttrNVMFlt]
  Ground172/1 -> [sTmIn_D_u8GrlShttrOvertravelErr]
  Ground173/1 -> [sTmIn_D_u8GrlShttrOverVolt]
  Ground174/1 -> [sTmIn_D_u8GrlShttrStsShttrActrFlt]
  Ground175/1 -> [sTmIn_D_u8GrlShttrStsShttrBlkd]
  Ground176/1 -> [sTmIn_D_u8GrlShttrStsShttrCalActv]
  Ground177/1 -> [sTmIn_D_u8GrlShttrStsShttrCalIndcd]
  Ground178/1 -> [sTmIn_D_u8GrlShttrStsShttrElecErr]
  Ground179/1 -> [sTmIn_Te_s32HvBattCooltTOut]
  Ground180/1 -> [sTmIn_D_u8GrlShttrStsShttrSnsrFlt]
  Ground181/1 -> [sTmIn_D_u8GrlShttrStsShttrTErr]
  Ground182/1 -> [sTmIn_D_u8GrlShttrStsShttrULoErr]
  Ground183/1 -> [sTmIn_X_s32GrlShttrStsShttrPosnRaw]
  Ground184/1 -> [sTmIn_D_u8CircForDrvrShoOrOpen]
  Ground185/1 -> [sTmIn_D_u8CooltTInSnsrFlt]
  Ground186/1 -> [sTmIn_D_u8CooltTOutOfRng]
  Ground187/1 -> [sTmIn_D_u8CooltTOutSnsrFlt]
  Ground188/1 -> [sTmIn_D_u8HeatrStsSig]
  Ground189/1 -> [sTmIn_D_u8HvOutOfRng]
  Ground190/1 -> [sTmIn_L_s32IsgCooltFlowMinReq]
  Ground191/1 -> [sTmIn_D_u8ICnsOutOfRng]
  Ground192/1 -> [sTmIn_D_u8MemErr]
  Ground193/1 -> [sTmIn_D_u8SelfTmpSigHwProtn]
  Ground194/1 -> [sTmIn_D_u8SelfTmpSigOvrheatg]
  Ground195/1 -> [sTmIn_D_u8TInMtrlSnsrFlt]
  Ground196/1 -> [sTmIn_D_u8ULoOutOfRng]
  Ground197/1 -> [sTmIn_Pw_s32HvHeatrPwrCns]
  Ground198/1 -> [sTmIn_Pw_s32HvHeatrPwrCnsDes]
  Ground199/1 -> [sTmIn_Te_s32WtrTInIntk]
  Ground200/1 -> [sTmIn_Te_s32WtrTInOutl]
  Ground201/1 -> [sTmIn_Te_s32Coolt]
  Ground202/1 -> [sTmIn_D_u8SrvRqrd]
  Ground203/1 -> [sTmIn_D_u8TmpSigProtnOfSelfTmp]
  Ground204/1 -> [sTmIn_D_u8HvCoolgCmd]
  Ground205/1 -> [sTmIn_D_u8HvHvacCmd]
  Ground206/1 -> [sTmIn_D_u8HvActvSts]
  Ground207/1 -> [sTmIn_D_u8PowerPackStatus]
  Ground208/1 -> [sTmIn_Pw_s32HvCoolgAllwd]
  Ground209/1 -> [sTmIn_Pw_s32HvHeatgAllwd]
  Ground210/1 -> [yTmIn_B_ElAcEnable]
  Ground211/1 -> [yTmIn_B_HvCooltHeatrEnad]
  Ground212/1 -> [sTmIn_D_u8HvgCoolReq]
  Ground213/1 -> [sTmIn_v_s32VehSpdLgt]
  Ground214/1 -> [yTmIn_B_StarDiagEval]
  Ground215/1 -> [sTmIn_D_u8HvActvReq]
  Ground216/1 -> [sTmIn_D_u8DCChrgSt]
  Ground217/1 -> [yTmIn_B_NOPCoolReq]
  Ground218/1 -> [sTmIn_Pw_s32HvBattChrgnPwrCritDes1]
  Ground219/1 -> [yTmIn_B_ChargePsr]
  Ground220/1 -> [sTmIn_Te_s32BattHvMin]
  Ground221/1 -> [sTmIn_D_u8HvBattSupChrgThermSts]
  Ground222/1 -> [sTmIn_D_u8OnBdChrgrSt]
  Ground223/1 -> [sTmIn_Te_s32EradInvActl]
  Ground224/1 -> [sTmIn_Te_s32HvgInvActl]
  Ground225/1 -> [sTmIn_D_u8DistHvBatt]
  Ground226/1 -> [sTmIn_D_u8ElecDriveline]
  Ground227/1 -> [sTmIn_D_u8HiWayAsst]
  Ground228/1 -> [sTmIn_D_u8CruiseCtrl]
  Ground229/1 -> [sTmIn_D_u8BattCntct]
  Ground230/1 -> [sTmIn_U_s32HvBattUDc]
  Ground231/1 -> [yTmIn_B_EvaprTFrntUD]
  Ground232/1 -> [sTmIn_Te_s32HmiCmptmtTSpForRowFirstRi]
  Ground233/1 -> [sTmIn_Te_s32HmiCmptmtTSpForRowFirstLe]
  Ground234/1 -> [sTmIn_D_u8HvUSplyErrSts]
  Ground235/1 -> [sTmIn_Te_s32HvgWndgActl]
  Ground236/1 -> [sTmIn_D_u8LnchModSts]
  Ground237/1 -> [sTmIn_D_u8LaunchCtrl]
  Ground238/1 -> [sTmIn_X_s32HvacTFlpActlPosnFrtRowLe]
  Ground239/1 -> [sTmIn_X_s32HvacTFlpActlPosnFrtRowRi]
  Ground240/1 -> [sTmIn_D_u8HmiCmptmtTSpSpclForRowFirstLe]
  Ground241/1 -> [sTmIn_D_u8HmiCmptmtTSpSpclForRowFirstRi]
  Ground242/1 -> [sTmIn_D_u8SysQf]
  Ground243/1 -> [yTmIn_B_ErrRespHVCH]
  Ground244/1 -> [sTmIn_I_s32HeatrICnsSig]
  Ground245/1 -> [sTmIn_D_u8HeatrInfoCompProtn]
  Ground246/1 -> [sTmIn_D_u8EngCooltLvl]
  Ground247/1 -> [sTmIn_U_u8SplyUForCtrlUnitVal]
  Ground248/1 -> [sTmIn_D_u8SelfSigProOfTmpResd]
  Ground249/1 -> [sTmIn_D_u8ResdForSnsrFlt]
  Ground250/1 -> [sTmIn_D_u8SrvRqrdResd]
  Ground251/1 -> [sTmIn_D_u8FltInComHVCH]
  Ground252/1 -> [sTmIn_D_u8FltPrsnt]
  Ground253/1 -> [sTmIn_D_u8FltPrsntResd]
  Ground254/1 -> [yTmIn_B_EctvComFault]
  Ground255/1 -> [sTmIn_D_u8EctvPosSts]
  Ground256/1 -> [sTmIn_D_u8EctvRunSts]
  Ground257/1 -> [sTmIn_U_s32Sys]
  Ground258/1 -> [sTmIn_D_u8EctvSpdLvl]
  Ground259/1 -> [yTmIn_B_BctvComFault]
  Ground260/1 -> [sTmIn_D_u8BctvVlvMode]
  Ground261/1 -> [sTmIn_D_u8BctvRunSts]
  Ground262/1 -> [sTmIn_D_u8BctvSpdLvl]
  Ground263/1 -> [yTmIn_B_BcfvComFault]
  Ground264/1 -> [sTmIn_D_u8BcfvVlvMode]
  Ground265/1 -> [sTmIn_X_s32BcfvPosSts]
  Ground266/1 -> [sTmIn_D_u8BcfvRunSts]
  Ground267/1 -> [sTmIn_D_u8BcfvSpdLvl]
  Ground268/1 -> [sTmIn_D_u8UsgModSts1WdSts]
  Ground269/1 -> [sTmIn_D_u8ErrRespACCM]
  Ground270/1 -> [sTmIn_D_u8SpdErrSts]
  Ground271/1 -> [sTmIn_D_u8CtrlrErrSts]
  Ground272/1 -> [sTmIn_D_u8AccmDrvrSircSnErrStsts]
  Ground273/1 -> [sTmIn_D_u8DrvrSircSnstPlausErrSts]
  Ground274/1 -> [sTmIn_D_u8AccmHvSnsrU1ErrSts]
  Ground275/1 -> [sTmIn_D_u8AccmHvSnsrU2ErrSts]
  Ground276/1 -> [sTmIn_D_u8AccmHvSnsrIErrSts]
  Ground277/1 -> [sTmIn_D_u8AccmSnsrICrctErrSts]
  Ground278/1 -> [sTmIn_D_u8HvSnsrIPlausErrSts]
  Ground279/1 -> [sTmIn_D_u8LVPwrSplyErrSts]
  Ground280/1 -> [sTmIn_D_u8HvSnsrUPlausErrSts]
  Ground281/1 -> [sTmIn_D_u8AccmPhaseWireErrSts]
  Ground282/1 -> [sTmIn_D_u8AccmT1ErrSts]
  Ground283/1 -> [sTmIn_D_u8AccmT2ErrSts]
  Ground284/1 -> [sTmIn_D_u8AccmCmprTOperErr1]
  Ground285/1 -> [sTmIn_D_u8AccmCmprTOperErr2]
  Ground286/1 -> [sTmIn_D_u8TPlausErrSts]
  Ground287/1 -> [sTmIn_D_u8AccmLoUSplyErrSts]
  Ground288/1 -> [sTmIn_I_s32CmprFbCmprIPha]
  Ground289/1 -> [sTmIn_D_u8CmprSts2]
  Ground290/1 -> [sTmIn_Z_s32RoadIncln]
  Ground291/1 -> [sTmIn_Te_s32CmprT2]
  Ground292/1 -> [sTmIn_D_u8EEPROMFault]
  Ground293/1 -> [sTmIn_D_u8LostCommStat]
  Ground294/1 -> [sTmIn_D_u8CmprSpdIncrReq]
  Ground295/1 -> [sTmIn_D_u8BexvMovSts]
  Ground296/1 -> [yTmIn_B_CexvComFault]
  Ground297/1 -> [sTmIn_X_s32CexvPosSts]
  Ground298/1 -> [sTmIn_D_u8CexvCalibSts]
  Ground299/1 -> [sTmIn_D_u8CexvMovSts]
  Ground300/1 -> [sTmIn_D_u8CexvPreHeatgSts]
  Ground301/1 -> [sTmIn_D_u8CarModSts1]
  Ground302/1 -> [yTmIn_B_EexvComFault]
  Ground303/1 -> [sTmIn_X_s32EexvPosSts]
  Ground304/1 -> [sTmIn_D_u8EexvCalibSts]
  Ground305/1 -> [sTmIn_D_u8EexvMovSts]
  Ground306/1 -> [sTmIn_D_u8EexvPreHeatgSts]
  Ground307/1 -> [yTmIn_B_HvacHexAirTUD]
  Ground308/1 -> [yTmIn_B_EcoClimaSts]
  Ground309/1 -> [sTmIn_t_s32BattPmpPwmTHigh]
  Ground310/1 -> [yTmIn_B_BattPmpTHighValid]
  Ground311/1 -> [sTmIn_t_s32BattPmpPwmTLow]
  Ground312/1 -> [sTmIn_Te_s32AmbTEstimd]
  Ground313/1 -> [yTmIn_B_BattPmpTLowValid]
  Ground314/1 -> [sTmIn_t_s32EmotPmpPwmTHigh]
  Ground315/1 -> [yTmIn_B_EmotPmpTHighValid]
  Ground316/1 -> [sTmIn_t_s32EmotPmpPwmTLow]
  Ground317/1 -> [yTmIn_B_EmotPmpTLowValid]
  Ground318/1 -> [sTmIn_t_s32FanPwmTHigh]
  Ground319/1 -> [yTmIn_B_FanTHighValid]
  Ground320/1 -> [sTmIn_t_s32FanPwmTLow]
  Ground321/1 -> [yTmIn_B_FanTLowValid]
  Ground322/1 -> [sTmIn_t_s32HmPumpPwmTHigh]
  Ground323/1 -> [sTmIn_Te_s32Evap]
  Ground324/1 -> [yTmIn_B_HmPumpTHighValid]
  Ground325/1 -> [sTmIn_t_s32HmPumpPwmTLow]
  Ground326/1 -> [yTmIn_B_HmPumpTLowValid]
  Ground327/1 -> [sTmIn_D_u8HeatStopReq]
  Ground328/1 -> [yTmIn_B_AD4CoolReq]
  Ground329/1 -> [sTmIn_L_s32AD4CooltFlowReq]
  Ground330/1 -> [sTmIn_L_s32DHUCooltFlowMinReq]
  Ground331/1 -> [sTmIn_D_u8VcEvLoSidePOP]
  Ground332/1 -> [sTmIn_D_u8VcEvLoSidePSB]
  Ground333/1 -> [sTmIn_D_u8VcEvHiSidePOP]
  Ground334/1 -> [sTmIn_Te_s32EradWndgActl]
  Ground335/1 -> [sTmIn_Te_s32EvapReq]
  Ground336/1 -> [sTmIn_D_u8VcEvHiSidePSB]
  Ground337/1 -> [sTmIn_D_u8VcEvHiSideTmpSnrSG]
  Ground338/1 -> [sTmIn_D_u8VcEvOutrCondOutTOP]
  Ground339/1 -> [sTmIn_D_u8VcEvChillerOutTSG]
  Ground340/1 -> [sTmIn_D_u8VcEvChillerOutTOP]
  Ground341/1 -> [sTmIn_D_u8VcEvInrCondOutTSG]
  Ground342/1 -> [sTmIn_D_u8VcEvInrCondOutTOP]
  Ground343/1 -> [sTmIn_D_u8VcEvEvapOutTSG]
  Ground344/1 -> [sTmIn_D_u8VcEvEvapOutTOP]
  Ground345/1 -> [sTmIn_D_u8VcEvCmprDischrgTSG]
  Ground346/1 -> [sTmIn_Te_s32HeadEstimdFirstRow]
  Ground347/1 -> [sTmIn_D_u8VcEvCmprDischrgTOP]
  Ground348/1 -> [sTmIn_D_u8VcEvTmpClSrSG]
  Ground349/1 -> [sTmIn_D_u8VcEvTmpClSrOP]
  Ground350/1 -> [sTmIn_D_u8VcEvBattCooltLvlLo]
  Ground351/1 -> [sTmIn_D_u8VcEvNoHpHighSidePSnrOP]
  Ground352/1 -> [sTmIn_D_u8VcEvNoHpHighSidePSnrSB]
  Ground353/1 -> [sTmIn_D_u8VcEvSov1OP]
  Ground354/1 -> [sTmIn_D_u8VcEvSov1SB]
  Ground355/1 -> [sTmIn_D_u8VcEvSov1SG]
  Ground356/1 -> [sTmIn_D_u8VcEvSov2OP]
  Ground357/1 -> [sTmIn_Te_s32HeatrAirTReq]
  Ground358/1 -> [sTmIn_D_u8VcEvSov2SB]
  Ground359/1 -> [sTmIn_D_u8VcEvSov2SG]
  Ground360/1 -> [sTmIn_D_u8VcEvSov3OP]
  Ground361/1 -> [sTmIn_D_u8VcEvSov3SB]
  Ground362/1 -> [sTmIn_D_u8VcEvSov3SG]
  Ground363/1 -> [sTmIn_D_u8VcEvSov4OP]
  Ground364/1 -> [sTmIn_D_u8VcEvSov4SB]
  Ground365/1 -> [sTmIn_D_u8VcEvSov4SG]
  Ground366/1 -> [sTmIn_D_u8VcEvSov5OP]
  Ground367/1 -> [sTmIn_D_u8VcEvSov5SB]
  Ground368/1 -> [sTmIn_Te_s32HvacHexAirT]
  Ground369/1 -> [sTmIn_D_u8VcEvSov5SG]
  Ground370/1 -> [sTmIn_D_u8VcEvSBFan]
  Ground371/1 -> [sTmIn_D_u8VcEvSGFan]
  Ground372/1 -> [sTmIn_D_u8VcEvOPFan]
  Ground373/1 -> [sTmIn_D_u8VcEvFanOvrTShDwn]
  Ground374/1 -> [sTmIn_D_u8VcEvBlokFan]
  Ground375/1 -> [sTmIn_D_u8VcEvCircutInteFlt]
  Ground376/1 -> [sTmIn_D_u8VcEvVolErrFan]
  Ground377/1 -> [sTmIn_D_u8VcEvHmPumpSG]
  Ground378/1 -> [sTmIn_D_u8VcEvHmPumpSB]
  Ground379/1 -> [sTmIn_X_s32ClimtRcirc]
  Ground380/1 -> [sTmIn_D_u8VcEvHmPumpOC]
  Ground381/1 -> [sTmIn_D_u8VcEvHmPmpOvrTShutDwn]
  Ground382/1 -> [sTmIn_D_u8VcEvHmPmpStall]
  Ground383/1 -> [sTmIn_D_u8VcEvHmPmpVolErr]
  Ground384/1 -> [sTmIn_D_u8VcEvHmPmpDyRn]
  Ground385/1 -> [sTmIn_D_u8VcEvSGBatteryPmp]
  Ground386/1 -> [sTmIn_D_u8VcEvSBBatteryPmp]
  Ground387/1 -> [sTmIn_D_u8VcEvOCBatteryPmp]
  Ground388/1 -> [sTmIn_D_u8VcEvBattPmpOvrTShutDwn]
  Ground389/1 -> [sTmIn_D_u8VcEvBattPmpStall]
  Ground390/1 -> [sTmIn_md_s32HexHeatrAirMFlowEstimd]
  Ground391/1 -> [sTmIn_D_u8VcEvBattPmpVolErr]
  Ground392/1 -> [sTmIn_D_u8VcEvBattPmpDyn]
  Ground393/1 -> [sTmIn_D_u8VcEvSGEmotor]
  Ground394/1 -> [sTmIn_D_u8VcEvSBEmotor]
  Ground395/1 -> [sTmIn_D_u8VcEvOCEmotor]
  Ground396/1 -> [sTmIn_D_u8VcEvEmPmpOvrTShutDwn]
  Ground397/1 -> [sTmIn_D_u8VcEvEmPmpStall]
  Ground398/1 -> [sTmIn_D_u8VcEvEmPmpVolErr]
  Ground399/1 -> [sTmIn_D_u8VcEvEmPmpDyRn]
  Ground400/1 -> [sTmIn_D_u8VcEvBctvOthrErr]
  Ground401/1 -> [sTmIn_md_s32HvacAirMFlowEstimd]
  Ground402/1 -> [sTmIn_D_u8VcEvFltTemBCTV]
  Ground403/1 -> [sTmIn_D_u8VcEvBctvBlk]
  Ground404/1 -> [sTmIn_D_u8VcEvBctvErrResp]
  Ground405/1 -> [sTmIn_D_u8VcEvFltVolBCTV]
  Ground406/1 -> [sTmIn_D_u8VcEvBctvNVMFlt]
  Ground407/1 -> [sTmIn_D_u8VcEvBctvIniFail]
  Ground408/1 -> [sTmIn_D_u8VcEvBcfvOthrErr]
  Ground409/1 -> [sTmIn_D_u8VcEvFltTempBCFV]
  Ground410/1 -> [sTmIn_D_u8VcEvBcfvBlk]
  Ground411/1 -> [sTmIn_D_u8VcEvBcfvErrResp]
  Ground412/1 -> [yTmIn_B_AirCondEnbl]
  Ground413/1 -> [sTmIn_D_u8VcEvFltVolBCFV]
  Ground414/1 -> [sTmIn_D_u8VcEvBcfvNVMFlt]
  Ground415/1 -> [sTmIn_D_u8VcEvBcfvIniFail]
  Ground416/1 -> [sTmIn_D_u8VcEvEctvDrvMotorFlt]
  Ground417/1 -> [sTmIn_D_u8VcEvWarnECRV]
  Ground418/1 -> [sTmIn_D_u8VcEvEcrvErrResp]
  Ground419/1 -> [sTmIn_D_u8VcEvFltVolECRV]
  Ground420/1 -> [sTmIn_D_u8VcEvBexvIniFail]
  Ground421/1 -> [sTmIn_D_u8VcEvBexvOvrTempErr]
  Ground422/1 -> [sTmIn_D_u8VcEvBexvBlkErr]
  Ground423/1 -> [yTmIn_B_ClimaDefrstSts]
  Ground424/1 -> [sTmIn_D_u8VcEvBexvErrResp]
  Ground425/1 -> [sTmIn_D_u8VcEvBexvVoltgRangErr]
  Ground426/1 -> [sTmIn_D_u8VcEvBexvNVMFlt]
  Ground427/1 -> [sTmIn_D_u8VcEvCexvIniFail]
  Ground428/1 -> [sTmIn_D_u8VcEvCexvOvrTempErr]
  Ground429/1 -> [sTmIn_D_u8VcEvCexvBlkErr]
  Ground430/1 -> [sTmIn_D_u8VcEvCexvErrResp]
  Ground431/1 -> [sTmIn_D_u8VcEvCexvVoltgRangErr]
  Ground432/1 -> [sTmIn_D_u8VcEvCexvNVMFlt]
  Ground433/1 -> [sTmIn_D_u8VcEvEexvIniFail]
  Ground434/1 -> [yTmIn_B_HvacHeatgReq]
  Ground435/1 -> [sTmIn_D_u8VcEvEexvOvrTempErr]
  Ground436/1 -> [sTmIn_D_u8VcEvEexvBlkErr]
  Ground437/1 -> [sTmIn_D_u8VcEvEexvErrResp]
  Ground438/1 -> [sTmIn_D_u8VcEvEexvVoltgRangErr]
  Ground439/1 -> [sTmIn_D_u8VcEvEexvNVMFlt]
  Ground440/1 -> [sTmIn_D_u8VcEvAccmUSplyErr]
  Ground441/1 -> [sTmIn_D_u8VcEvAccmOCFlt]
  Ground442/1 -> [sTmIn_D_u8VcEvAccmMotOvrCur]
  Ground443/1 -> [sTmIn_D_u8VcEvAccmComFlt]
  Ground444/1 -> [sTmIn_D_u8VcEvCurDrCirtACCM]
  Ground445/1 -> [sTmIn_Tq_s32WhlMotSysTqEst]
  Ground446/1 -> [sTmIn_Te_s32IncarTemp]
  Ground447/1 -> [sTmIn_D_u8VcEvAccmRotorLock]
  Ground448/1 -> [sTmIn_D_u8VcEvAccmOPFlt]
  Ground449/1 -> [sTmIn_D_u8VcEvLiquidSluggingACCM]
  Ground450/1 -> [sTmIn_D_u8VcEvMemFltAccm]
  Ground451/1 -> [sTmIn_D_u8VcEvTM_AGM_OVRTEMP]
  Ground452/1 -> [sTmIn_D_u8VcEvAgsBlk]
  Ground453/1 -> [sTmIn_D_u8VcEvAgsErrResp]
  Ground454/1 -> [sTmIn_D_u8VcEvAgsVoltErr]
  Ground455/1 -> [sTmIn_D_u8VcEvAgsMechErr]
  Ground456/1 -> [sTmIn_D_u8VcEvAgsNVMFlt]
  Ground457/1 -> [yTmIn_B_AmbTEstimdQf]
  Ground458/1 -> [sTmIn_D_u8VcEvAgsElecErr]
  Ground459/1 -> [sTmIn_D_u8VcEvIGBTSpOrOpHVCH]
  Ground460/1 -> [sTmIn_D_u8VcEvLoVoOvrHVCH]
  Ground461/1 -> [sTmIn_D_u8VcEvVolMemErrHVCH]
  Ground462/1 -> [sTmIn_D_u8VcEvComFltHVCH]
  Ground463/1 -> [sTmIn_D_u8VcEvHiVoOvrHVCH]
  Ground464/1 -> [sTmIn_D_u8VcEvCoolTempOutOfRng]
  Ground465/1 -> [sTmIn_D_u8VcEvTempSerIntHVCH]
  Ground466/1 -> [sTmIn_D_u8VcEvTempSerOutHVCH]
  Ground467/1 -> [sTmIn_D_u8VcEvHWProtHVCH]
  Ground468/1 -> [sTmIn_D_u8IncarTempQf]
  Ground469/1 -> [sTmIn_D_u8VcEvInterSerTempHVCH]
  Ground470/1 -> [sTmIn_D_u8VcEvCurrOutOfRng]
  Ground471/1 -> [sTmIn_D_u8LackRefrigerant]
  Ground472/1 -> [sTmIn_D_u8HvBoostMod]
  Ground473/1 -> [yTmIn_B_HmiMaxACReq]
  Ground474/1 -> [yTmIn_B_GrlShttrAutoCalibReq2FReq]
  Ground475/1 -> [yTmIn_B_GrlShttrAutoCalibReqReq2F]
  Ground476/1 -> [sTmIn_X_s32PTCPumpPwmFb]
  Ground477/1 -> [yTmIn_B_MessMissBctv]
  Ground478/1 -> [yTmIn_B_MessMissBCFV]
  Ground479/1 -> [yTmIn_B_HvacOsaAndRecActrQfForHp]
  Ground480/1 -> [yTmIn_B_MessMissECRV]
  Ground481/1 -> [yTmIn_B_MessMissBEXV]
  Ground482/1 -> [yTmIn_B_MessMissCEXV]
  Ground483/1 -> [yTmIn_B_MessMissEEXV]
  Ground484/1 -> [yTmIn_B_MessMissAccm]
  Ground485/1 -> [yTmIn_B_MessMissAGM]
  Ground486/1 -> [yTmIn_B_MessMissHVCH]
  Ground487/1 -> [sTmIn_Tq_s32TotAxle]
  Ground488/1 -> [sTmIn_Z_s32HvacModResp]
  Ground489/1 -> [sTmIn_Te_s32HvBattTAvg]
  Ground490/1 -> [yTmIn_B_TeEvap]
  Ground491/1 -> [yTmIn_B_AD4CoolReqForBkp]
  Ground492/1 -> [sTmIn_L_s32AD4CooltFlowReqForBkp]
  Ground493/1 -> [yTmIn_B_ChillerValveReqFb]
  Ground494/1 -> [yTmIn_B_EvaprVlvReqFrntFb]
  Ground495/1 -> [yTmIn_B_HpmSov1ActvCmdFb]
  Ground496/1 -> [yTmIn_B_HpmSov2ActvCmdFb]
  Ground497/1 -> [yTmIn_B_HpmSov3ActvCmdFb]
  Ground498/1 -> [yTmIn_B_EmActivHeatAllwd]
  Ground499/1 -> [sTmIn_D_u8IsgHeatFdBck]
  Ground500/1 -> [sTmIn_D_u8WhlMotSysHeatFdBck]
  Ground501/1 -> [yTmIn_B_HvacHexAirTQf]
  Ground502/1 -> [sTmIn_Pw_s32IsgHeatPwrAct]
  Ground503/1 -> [sTmIn_Pw_s32WhlMotSysHeatPwrAct]
  Ground504/1 -> [sTmIn_Pw_s32ElecDrvHeatgPwrAllwd]
  Ground505/1 -> [sTmIn_Pw_s32WhlMotSysHeatPwrMax]
  Ground506/1 -> [sTmIn_Pw_s32IsgHeatPwrMax]
  Ground507/1 -> [sTmIn_X_s32BattCooltPmpPwmFb]
  Ground508/1 -> [sTmIn_D_u8CmprSupplrNo]
  Ground509/1 -> [sTmIn_D_u8VcEvEctvBlk]
  Ground510/1 -> [sTmIn_D_u8VcEvOVACCM]
  Ground511/1 -> [sTmIn_D_u8VcEvAccmIgbtOvrTErr]
  Ground512/1 -> [sTmIn_D_u8HvacFanSts]
  Ground513/1 -> [sTmIn_D_u8VcEvAccmSnsrFlt]
  Ground514/1 -> [sTmIn_D_u8VcEvAccmPhaseFail]
  Ground515/1 -> [yTmIn_B_AD4CoolReqForBkpUD]
  Ground516/1 -> [yTmIn_B_AD4CoolReqUD]
  Ground517/1 -> [yTmIn_B_AD4CooltFlowReqForBkpUD]
  Ground518/1 -> [yTmIn_B_AD4CooltFlowReqUD]
  Ground519/1 -> [sTmIn_D_u8VcEvOvrTempHVCH]
  Ground520/1 -> [sTmIn_B_HvBattLimnIndcnUD]
  Ground521/1 -> [yTmIn_B_ImpactDetect]
  Ground522/1 -> [yTmIn_B_BattPmpOPflg]
  Ground523/1 -> [yTmIn_B_BattPmpOPTF]
  Ground524/1 -> [sTmIn_D_u8DcdcCoolReq]
  Ground525/1 -> [yTmIn_B_BattPmpSBflg]
  Ground526/1 -> [yTmIn_B_BattPmpSBTF]
  Ground527/1 -> [yTmIn_B_BattPmpSGflg]
  Ground528/1 -> [yTmIn_B_BattPmpSGTF]
  Ground529/1 -> [yTmIn_B_EmotPmpOPflg]
  Ground530/1 -> [yTmIn_B_EmotPmpOPTF]
  Ground531/1 -> [yTmIn_B_EmotPmpSBflg]
  Ground532/1 -> [yTmIn_B_EmotPmpSBTF]
  Ground533/1 -> [yTmIn_B_EmotPmpSGflg]
  Ground534/1 -> [yTmIn_B_EmotPmpSGTF]
  Ground535/1 -> [sTmIn_Te_s32DcdcActl]
  Ground536/1 -> [yTmIn_B_FanOutOPflg]
  Ground537/1 -> [yTmIn_B_FanOutOPTF]
  Ground538/1 -> [yTmIn_B_FanOutSBflg]
  Ground539/1 -> [yTmIn_B_FanOutSBTF]
  Ground540/1 -> [yTmIn_B_FanOutSGflg]
  Ground541/1 -> [yTmIn_B_FanOutSGTF]
  Ground542/1 -> [yTmIn_B_HmPumpOCflg]
  Ground543/1 -> [yTmIn_B_HmPumpOCTF]
  Ground544/1 -> [yTmIn_B_HmPumpSBflg]
  Ground545/1 -> [yTmIn_B_HmPumpSBTF]
  Ground546/1 -> [sTmIn_L_s32DcDcMinCooltFlow]
  Ground547/1 -> [yTmIn_B_HmPumpSGflg]
  Ground548/1 -> [yTmIn_B_HmPumpSGTF]
  Ground549/1 -> [yTmIn_B_Sov1OPTF]
  Ground550/1 -> [yTmIn_B_Sov1OPflg]
  Ground551/1 -> [yTmIn_B_Sov1SBTF]
  Ground552/1 -> [yTmIn_B_Sov1SBflg]
  Ground553/1 -> [yTmIn_B_Sov1SGTF]
  Ground554/1 -> [yTmIn_B_Sov1SGflg]
  Ground555/1 -> [yTmIn_B_Sov2OPTF]
  Ground556/1 -> [yTmIn_B_Sov2OPflg]
  Ground557/1 -> [sTmIn_D_u8ObcCoolReq]
  Ground558/1 -> [yTmIn_B_Sov2SBTF]
  Ground559/1 -> [yTmIn_B_Sov2SBflg]
  Ground560/1 -> [yTmIn_B_Sov2SGTF]
  Ground561/1 -> [yTmIn_B_Sov2SGflg]
  Ground562/1 -> [yTmIn_B_Sov3OPTF]
  Ground563/1 -> [yTmIn_B_Sov3OPflg]
  Ground564/1 -> [yTmIn_B_Sov3SBTF]
  Ground565/1 -> [yTmIn_B_Sov3SBflg]
  Ground566/1 -> [yTmIn_B_Sov3SGTF]
  Ground567/1 -> [yTmIn_B_Sov3SGflg]
